simulink model "KUKA_Linear"  (R2020b)
settings: Solver=VariableStepAuto  StartTime=0.0  StopTime=200  RelTol=1e-3
(part 1 of 3)
settings Model: Creator=amin1  LastModifiedBy=amin1

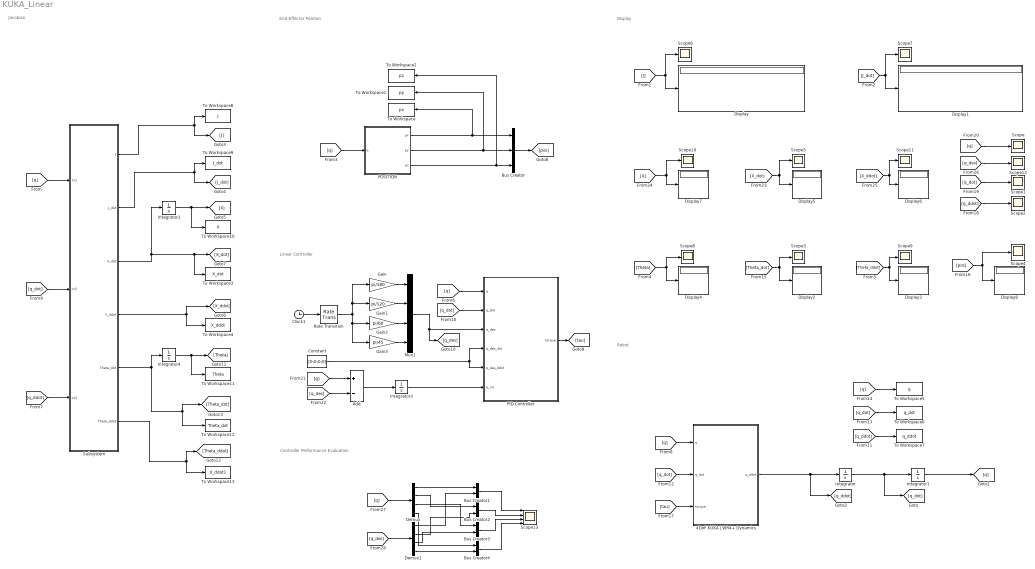
== system KUKA_Linear ==
  note: Controller Performance Evaluation
  note: Jacobian
  note: Display
  note: End-Effector Position
  note: Linear Controller
  note: Robot
  " 4DoF KUKA LWR4+ Dynamics" : MATLAB Function  TreatAsAtomicUnit=on
  Add : Sum  Inputs=+-
  Bus Creator : BusCreator  Inputs=3
  Bus Creator{1..4} (4 alike) : BusCreator  Inputs=2
  Clock1 : Clock
  Constant : Constant  Value=[0;0;0;0]
  Demux : Demux
  Demux1 : Demux
  Display{,1..8} (9 alike) : Display
  Gain : Gain  Gain=pi/180
  Gain1 : Gain  Gain=pi/120
  Gain2 : Gain  Gain=pi/60
  Gain3 : Gain  Gain=pi/45
  Integrator : Integrator  InitialCondition=[0;0;0;0]
  Integrator1 : Integrator  InitialCondition=[1;1;1;1]
  Integrator2 : Integrator  InitialCondition=[-0.458;-0.202;0.479]
  Integrator3 : Integrator  InitialCondition=[0;0;0;0]
  Integrator4 : Integrator  InitialCondition=[-0.455;-0.19;0.48]
  Mux1 : Mux
  PID Controller : MATLAB Function  TreatAsAtomicUnit=on
  POSITION : MATLAB Function  TreatAsAtomicUnit=on
  Rate Transition : RateTransition  OutPortSampleTime=10
  Scope{,1..12} (13 alike) : Scope
  Scope13 : Scope  NumInputPorts=4
  Subsystem : Subsystem
  To Workspace : ToWorkspace  VariableName=px  SampleTime=-1
  To Workspace1 : ToWorkspace  VariableName=py  SampleTime=-1
  To Workspace10 : ToWorkspace  VariableName=X  SampleTime=-1
  To Workspace11 : ToWorkspace  VariableName=Theta  SampleTime=-1
  To Workspace12 : ToWorkspace  VariableName=Theta_dot  SampleTime=-1
  To Workspace13 : ToWorkspace  VariableName=X_ddot1  SampleTime=-1
  To Workspace2 : ToWorkspace  VariableName=pz  SampleTime=-1
  To Workspace3 : ToWorkspace  VariableName=X_dot  SampleTime=-1
  To Workspace4 : ToWorkspace  VariableName=X_ddot  SampleTime=-1
  To Workspace5 : ToWorkspace  VariableName=q  SampleTime=-1
  To Workspace6 : ToWorkspace  VariableName=q_dot  SampleTime=-1
  To Workspace7 : ToWorkspace  VariableName=q_ddot  SampleTime=-1
  To Workspace8 : ToWorkspace  VariableName=J  SampleTime=-1
  To Workspace9 : ToWorkspace  VariableName=J_dot  SampleTime=-1
  wires:
  Gain/1 -> Mux1/1
  [q_dot] -> To Workspace6/1
  [q] -> To Workspace5/1
  POSITION/2(py) -> Bus Creator/2, To Workspace1/1
  Mux1/1 -> PID Controller/3(q_des), [q_des]
  Gain2/1 -> Mux1/3
  [q_dot] -> PID Controller/2(q_dot)
  [q_ddot] -> To Workspace7/1
  POSITION/3(pz) -> Bus Creator/3, To Workspace2/1
  Clock1/1 -> Rate Transition/1
  Constant/1 -> PID Controller/5(q_des_ddot), PID Controller/4(q_des_dot)
  [q] -> POSITION/1(q)
  [q] -> PID Controller/1(q)
  Rate Transition/1 -> Gain1/1, Gain/1, Gain2/1, Gain3/1
  " 4DoF KUKA LWR4+ Dynamics"/1(q_ddot) -> Integrator/1, [q_ddot]
  [q] -> " 4DoF KUKA LWR4+ Dynamics"/1(q)
  [q_dot] -> " 4DoF KUKA LWR4+ Dynamics"/2(q_dot)
  POSITION/1(px) -> Bus Creator/1, To Workspace/1
  Gain1/1 -> Mux1/2
  Integrator/1 -> Integrator1/1, [q_dot]
  Integrator1/1 -> [q]
  Gain3/1 -> Mux1/4
  Subsystem/2(J_dot) -> [J_dot], To Workspace9/1
  Subsystem/3(X_dot) -> Integrator2/1, To Workspace3/1, [X_dot]
  Subsystem/1(J) -> [J], To Workspace8/1
  [q] -> Subsystem/1(In1)
  [q_ddot] -> Subsystem/3(In3)
  [q_dot] -> Subsystem/2(In2)
  Subsystem/4(X_ddot) -> To Workspace4/1, [X_ddot]
  Integrator2/1 -> To Workspace10/1, [X]
  [J] -> Display/1, Scope6/1
  [J_dot] -> Display1/1, Scope7/1
  [Theta] -> Display4/1, Scope8/1
  [Theta_dot] -> Display2/1, Scope3/1
  [Theta_ddot] -> Display3/1, Scope9/1
  Bus Creator/1 -> [pos]
  [pos] -> Display8/1, Scope4/1
  PID Controller/1(torque) -> [tau]
  [tau] -> " 4DoF KUKA LWR4+ Dynamics"/3(torque)
  [q_ddot] -> Scope2/1
  [q_dot] -> Scope1/1
  [q] -> Scope/1
  [q] -> Add/1
  [q_des] -> Add/2
  Add/1 -> Integrator3/1
  Integrator3/1 -> PID Controller/6(e_int)
  Subsystem/5(Theta_dot) -> [Theta_dot], To Workspace12/1, Integrator4/1
  Integrator4/1 -> To Workspace11/1, [Theta]
  Subsystem/6(Theta_ddot) -> [Theta_ddot], To Workspace13/1
  [X_ddot] -> Display6/1, Scope11/1
  [X_dot] -> Display5/1, Scope5/1
  [X] -> Display7/1, Scope10/1
  [q_des] -> Scope12/1
  [q] -> Demux/1
  [q_des] -> Demux1/1
  Demux/1 -> Bus Creator1/1
  Demux1/1 -> Bus Creator1/2
  Demux/2 -> Bus Creator2/1
  Demux1/2 -> Bus Creator2/2
  Demux/3 -> Bus Creator3/1
  Demux1/3 -> Bus Creator3/2
  Demux/4 -> Bus Creator4/1
  Demux1/4 -> Bus Creator4/2
  Bus Creator1/1 -> Scope13/1
  Bus Creator2/1 -> Scope13/2
  Bus Creator3/1 -> Scope13/3
  Bus Creator4/1 -> Scope13/4

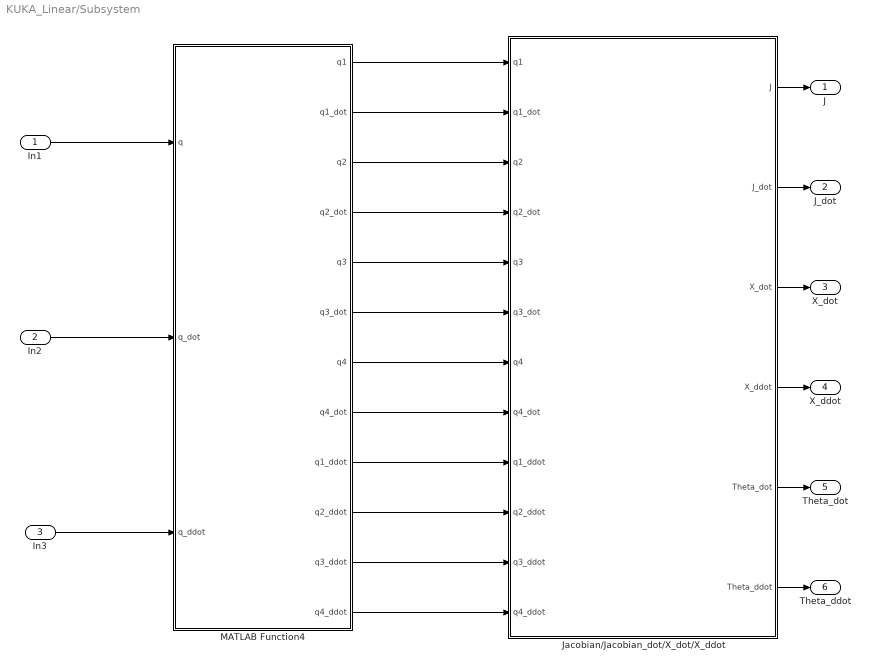
== system KUKA_Linear/Subsystem ==
  In1 : Inport
  In2 : Inport  Port=2
  In3 : Inport  Port=3
  Jacobian/Jacobian_dot/X_dot/X_ddot : MATLAB Function  TreatAsAtomicUnit=on
  MATLAB Function4 : MATLAB Function  TreatAsAtomicUnit=on
  J : Outport
  J_dot : Outport  Port=2
  X_dot : Outport  Port=3
  X_ddot : Outport  Port=4
  Theta_dot : Outport  Port=5
  Theta_ddot : Outport  Port=6
  wires:
  In2/1 -> MATLAB Function4/2(q_dot)
  In3/1 -> MATLAB Function4/3(q_ddot)
  In1/1 -> MATLAB Function4/1(q)
  MATLAB Function4/3(q2) -> Jacobian/Jacobian_dot/X_dot/X_ddot/3(q2)
  MATLAB Function4/10(q2_ddot) -> Jacobian/Jacobian_dot/X_dot/X_ddot/10(q2_ddot)
  MATLAB Function4/4(q2_dot) -> Jacobian/Jacobian_dot/X_dot/X_ddot/4(q2_dot)
  MATLAB Function4/11(q3_ddot) -> Jacobian/Jacobian_dot/X_dot/X_ddot/11(q3_ddot)
  MATLAB Function4/2(q1_dot) -> Jacobian/Jacobian_dot/X_dot/X_ddot/2(q1_dot)
  MATLAB Function4/1(q1) -> Jacobian/Jacobian_dot/X_dot/X_ddot/1(q1)
  MATLAB Function4/5(q3) -> Jacobian/Jacobian_dot/X_dot/X_ddot/5(q3)
  MATLAB Function4/6(q3_dot) -> Jacobian/Jacobian_dot/X_dot/X_ddot/6(q3_dot)
  MATLAB Function4/9(q1_ddot) -> Jacobian/Jacobian_dot/X_dot/X_ddot/9(q1_ddot)
  Jacobian/Jacobian_dot/X_dot/X_ddot/1(J) -> J/1
  Jacobian/Jacobian_dot/X_dot/X_ddot/2(J_dot) -> J_dot/1
  Jacobian/Jacobian_dot/X_dot/X_ddot/3(X_dot) -> X_dot/1
  Jacobian/Jacobian_dot/X_dot/X_ddot/4(X_ddot) -> X_ddot/1
  MATLAB Function4/7(q4) -> Jacobian/Jacobian_dot/X_dot/X_ddot/7(q4)
  MATLAB Function4/8(q4_dot) -> Jacobian/Jacobian_dot/X_dot/X_ddot/8(q4_dot)
  MATLAB Function4/12(q4_ddot) -> Jacobian/Jacobian_dot/X_dot/X_ddot/12(q4_ddot)
  Jacobian/Jacobian_dot/X_dot/X_ddot/6(Theta_ddot) -> Theta_ddot/1
  Jacobian/Jacobian_dot/X_dot/X_ddot/5(Theta_dot) -> Theta_dot/1

== matlab function KUKA_Linear/PID Controller ==
  data: q input; q_dot input; q_des input; torque output; q_des_dot input; q_des_ddot input; e_int input
function torque = fcn(q,q_dot,q_des,q_des_dot,q_des_ddot,e_int)
%#codegen

%% parameters
td1 = q_dot(1);
td2 = q_dot(2);
td3 = q_dot(3);
td4 = q_dot(4);

%% Constant
d3 = 0.4;

m1 = 2.7;
m2 = 2.7;
m3 = 2.7;
m4 = 2.7;

cx1 = 0.001340;
cx2 = 0.001340;
cx3 = -0.001340;
cx4 = -0.001340;

cy1 = -0.87777;
cy2 = -0.02622;
cy3 = 0.87777;
cy4 = 0.02622;

cz1 = -0.02622;
cz2 = 0.87777;
cz3 = -0.02622;
cz4 = 0.87777;

g = 9.8;

Ixx1 = 0.039; 
Ixy1 = 3.206e-4;
Ixz1 = 9.415e-5;
Iyy1 = 6.887e-3;
Iyz1 = -2.681e-3;
Izz1 = 0.03698;

Ixx2 = 0.039; 
Ixy2 = 9.415e-5;
Ixz2 = -3.145e-4;
Iyy2 = 0.03698;
Iyz2 = 9.747e-3;
Izz2 = 6.887e-3;

Ixx3 = 6.887e-3; 
Ixy3 = 3.145e-4;
Ixz3 = -9.5572e-5;
Iyy3 = 6.8872e-3;
Iyz3 = 2.681e-3;
Izz3 = 0.037;

Ixx4 = 0.037; 
Ixy4 = 9.415e-5;
Ixz4 = 3.1455e-4;
Iyy4 = 0.037;
Iyz4 = 9.747e-3;
Izz4 = 6.887e-3;

%% Triangle relative

c1 = cos(q(1));
c2 = cos(q(2));
c3 = cos(q(3));
c4 = cos(q(4)); 

s1 = sin(q(1));
s2 = sin(q(2));
s3 = sin(q(3));
s4 = sin(q(4));

%% matrix M

m11 = m1*cx1^2 + m1*cy1^2 + Izz1 - Iyz2*c2 - Ixz2*s2 - s2*(Ixz3*c2 + c3*(Ixx4*(c2*s4 - c3*c4*s2) - Ixy4*(c2*c4 + c3*s2*s4) + cy4*m4*(cy4*(c2*s4 - c3*c4*s2) - cx4*(c2*c4 + c3*s2*s4) + c3*d3*s2) + cz4*m4*(cz4*(c2*s4 - c3*c4*s2) - cx4*s2*s3 + d3*s2*s3*s4) - Ixz4*s2*s3) + s3*(Ixy4*(c2*s4 - c3*c4*s2) - Iyy4*(c2*c4 + c3*s2*s4) + cx4*m4*(cy4*(c2*s4 - c3*c4*s2) - cx4*(c2*c4 + c3*s2*s4) + c3*d3*s2) - cz4*m4*(cz4*(c2*c4 + c3*s2*s4) - cy4*s2*s3 + c4*d3*s2*s3) + Iyz4*s2*s3) - d3*m4*(cy4*(c2*s4 - c3*c4*s2) - cx4*(c2*c4 + c3*s2*s4) + c3*d3*s2) + cz3*m3*(c2*cx3 - c3*cz3*s2) - Ixx3*c3*s2 - Ixy3*s2*s3 - cy3*m3*(c3*cy3*s2 + cx3*s2*s3)) - c2*(Iyz3*c2 + d3*(c3*m4*(cz4*(c2*c4 + c3*s2*s4) - cy4*s2*s3 + c4*d3*s2*s3) + m4*s3*(cz4*(c2*s4 - c3*c4*s2) - cx4*s2*s3 + d3*s2*s3*s4)) - Ixz4*(c2*s4 - c3*c4*s2) - Iyz4*(c2*c4 + c3*s2*s4) - cy4*m4*(cz4*(c2*c4 + c3*s2*s4) - cy4*s2*s3 + c4*d3*s2*s3) - cx4*m4*(cz4*(c2*s4 - c3*c4*s2) - cx4*s2*s3 + d3*s2*s3*s4) + cz3*m3*(c2*cy3 + cz3*s2*s3) + Ixy3*c3*s2 + Iyy3*s2*s3 + Izz4*s2*s3 + cx3*m3*(c3*cy3*s2 + cx3*s2*s3)) - cx2*cz2*m2*s2 - c2*cy2*cz2*m2;
m12 = m2*cx2^2 + m2*cy2^2 + Izz2 - c2*(c3*m3*cz3^2 - d3*(c3*m4*(c3*cy4 - c3*c4*d3 + cz4*s3*s4) - m4*s3*(c4*cz4*s3 - c3*cx4 + c3*d3*s4)) + Iyy3*c3 + Izz4*c3 - Ixy3*s3 - Ixz4*c4*s3 + Iyz4*s3*s4 - cx4*m4*(c4*cz4*s3 - c3*cx4 + c3*d3*s4) + cy4*m4*(c3*cy4 - c3*c4*d3 + cz4*s3*s4) + cx3*m3*(c3*cx3 - cy3*s3)) - s2*(m3*s3*cz3^2 - Ixy3*c3 + Ixx3*s3 + c3*(cy4*m4*(c4*cy4*s3 - d3*s3 + cx4*s3*s4) - Ixz4*c3 + Ixx4*c4*s3 + Ixy4*s3*s4 + cz4*m4*(c4*cz4*s3 - c3*cx4 + c3*d3*s4)) + s3*(Iyz4*c3 + cx4*m4*(c4*cy4*s3 - d3*s3 + cx4*s3*s4) + Ixy4*c4*s3 + Iyy4*s3*s4 + cz4*m4*(c3*cy4 - c3*c4*d3 + cz4*s3*s4)) - d3*m4*(c4*cy4*s3 - d3*s3 + cx4*s3*s4) - cy3*m3*(c3*cx3 - cy3*s3));
m13 = c2*(Iyz4*c4 - Iyz3 + Ixz4*s4 - d3*(cz4*m4*s3*s4 + c3*c4*cz4*m4) - cy3*cz3*m3 + cx4*cz4*m4*s4 + c4*cy4*cz4*m4) - s2*(Ixz3 - c3*(- m4*s4*cz4^2 + Ixy4*c4 - Ixx4*s4 + cy4*m4*(c4*cx4 - cy4*s4)) - s3*(c4*m4*cz4^2 + Iyy4*c4 - Ixy4*s4 + cx4*m4*(c4*cx4 - cy4*s4)) + cx3*cz3*m3 + d3*m4*(c4*cx4 - cy4*s4));
m14 = s2*(s3*(Iyz4 + cy4*cz4*m4) - c3*(Ixz4 + cx4*cz4*m4)) + c2*(Izz4 - d3*(c3*cy4*m4 + cx4*m4*s3) + cx4^2*m4 + cy4^2*m4);

m21 = - Iyz2*c2 - Ixz2*s2 - s2*(Ixz3*c2 + c3*(Ixx4*(c2*s4 - c3*c4*s2) - Ixy4*(c2*c4 + c3*s2*s4) + cy4*m4*(cy4*(c2*s4 - c3*c4*s2) - cx4*(c2*c4 + c3*s2*s4) + c3*d3*s2) + cz4*m4*(cz4*(c2*s4 - c3*c4*s2) - cx4*s2*s3 + d3*s2*s3*s4) - Ixz4*s2*s3) + s3*(Ixy4*(c2*s4 - c3*c4*s2) - Iyy4*(c2*c4 + c3*s2*s4) + cx4*m4*(cy4*(c2*s4 - c3*c4*s2) - cx4*(c2*c4 + c3*s2*s4) + c3*d3*s2) - cz4*m4*(cz4*(c2*c4 + c3*s2*s4) - cy4*s2*s3 + c4*d3*s2*s3) + Iyz4*s2*s3) - d3*m4*(cy4*(c2*s4 - c3*c4*s2) - cx4*(c2*c4 + c3*s2*s4) + c3*d3*s2) + cz3*m3*(c2*cx3 - c3*cz3*s2) - Ixx3*c3*s2 - Ixy3*s2*s3 - cy3*m3*(c3*cy3*s2 + cx3*s2*s3)) - c2*(Iyz3*c2 + d3*(c3*m4*(cz4*(c2*c4 + c3*s2*s4) - cy4*s2*s3 + c4*d3*s2*s3) + m4*s3*(cz4*(c2*s4 - c3*c4*s2) - cx4*s2*s3 + d3*s2*s3*s4)) - Ixz4*(c2*s4 - c3*c4*s2) - Iyz4*(c2*c4 + c3*s2*s4) - cy4*m4*(cz4*(c2*c4 + c3*s2*s4) - cy4*s2*s3 + c4*d3*s2*s3) - cx4*m4*(cz4*(c2*s4 - c3*c4*s2) - cx4*s2*s3 + d3*s2*s3*s4) + cz3*m3*(c2*cy3 + cz3*s2*s3) + Ixy3*c3*s2 + Iyy3*s2*s3 + Izz4*s2*s3 + cx3*m3*(c3*cy3*s2 + cx3*s2*s3)) - cx2*cz2*m2*s2 - c2*cy2*cz2*m2;
m22 = m2*cx2^2 + m2*cy2^2 + Izz2 - c2*(c3*m3*cz3^2 - d3*(c3*m4*(c3*cy4 - c3*c4*d3 + cz4*s3*s4) - m4*s3*(c4*cz4*s3 - c3*cx4 + c3*d3*s4)) + Iyy3*c3 + Izz4*c3 - Ixy3*s3 - Ixz4*c4*s3 + Iyz4*s3*s4 - cx4*m4*(c4*cz4*s3 - c3*cx4 + c3*d3*s4) + cy4*m4*(c3*cy4 - c3*c4*d3 + cz4*s3*s4) + cx3*m3*(c3*cx3 - cy3*s3)) - s2*(m3*s3*cz3^2 - Ixy3*c3 + Ixx3*s3 + c3*(cy4*m4*(c4*cy4*s3 - d3*s3 + cx4*s3*s4) - Ixz4*c3 + Ixx4*c4*s3 + Ixy4*s3*s4 + cz4*m4*(c4*cz4*s3 - c3*cx4 + c3*d3*s4)) + s3*(Iyz4*c3 + cx4*m4*(c4*cy4*s3 - d3*s3 + cx4*s3*s4) + Ixy4*c4*s3 + Iyy4*s3*s4 + cz4*m4*(c3*cy4 - c3*c4*d3 + cz4*s3*s4)) - d3*m4*(c4*cy4*s3 - d3*s3 + cx4*s3*s4) - cy3*m3*(c3*cx3 - cy3*s3));
m23 = c2*(Iyz4*c4 - Iyz3 + Ixz4*s4 - d3*(cz4*m4*s3*s4 + c3*c4*cz4*m4) - cy3*cz3*m3 + cx4*cz4*m4*s4 + c4*cy4*cz4*m4) - s2*(Ixz3 - c3*(- m4*s4*cz4^2 + Ixy4*c4 - Ixx4*s4 + cy4*m4*(c4*cx4 - cy4*s4)) - s3*(c4*m4*cz4^2 + Iyy4*c4 - Ixy4*s4 + cx4*m4*(c4*cx4 - cy4*s4)) + cx3*cz3*m3 + d3*m4*(c4*cx4 - cy4*s4));
m24 = s2*(s3*(Iyz4 + cy4*cz4*m4) - c3*(Ixz4 + cx4*cz4*m4)) + c2*(Izz4 - d3*(c3*cy4*m4 + cx4*m4*s3) + cx4^2*m4 + cy4^2*m4);

m31 = Izz3*c2 - c3*(Ixy4*(c2*s4 - c3*c4*s2) - Iyy4*(c2*c4 + c3*s2*s4) + cx4*m4*(cy4*(c2*s4 - c3*c4*s2) - cx4*(c2*c4 + c3*s2*s4) + c3*d3*s2) - cz4*m4*(cz4*(c2*c4 + c3*s2*s4) - cy4*s2*s3 + c4*d3*s2*s3) + Iyz4*s2*s3) + s3*(Ixx4*(c2*s4 - c3*c4*s2) - Ixy4*(c2*c4 + c3*s2*s4) + cy4*m4*(cy4*(c2*s4 - c3*c4*s2) - cx4*(c2*c4 + c3*s2*s4) + c3*d3*s2) + cz4*m4*(cz4*(c2*s4 - c3*c4*s2) - cx4*s2*s3 + d3*s2*s3*s4) - Ixz4*s2*s3) + cx3*m3*(c2*cx3 - c3*cz3*s2) + cy3*m3*(c2*cy3 + cz3*s2*s3) - Ixz3*c3*s2 + Iyz3*s2*s3;
m32 = Iyz3*c3 + Ixz3*s3 - c3*(Iyz4*c3 + cx4*m4*(c4*cy4*s3 - d3*s3 + cx4*s3*s4) + Ixy4*c4*s3 + Iyy4*s3*s4 + cz4*m4*(c3*cy4 - c3*c4*d3 + cz4*s3*s4)) + s3*(cy4*m4*(c4*cy4*s3 - d3*s3 + cx4*s3*s4) - Ixz4*c3 + Ixx4*c4*s3 + Ixy4*s3*s4 + cz4*m4*(c4*cz4*s3 - c3*cx4 + c3*d3*s4)) + cx3*cz3*m3*s3 + c3*cy3*cz3*m3;
m33 = m3*cx3^2 + m3*cy3^2 + Izz3 + c3*(c4*m4*cz4^2 + Iyy4*c4 - Ixy4*s4 + cx4*m4*(c4*cx4 - cy4*s4)) - s3*(- m4*s4*cz4^2 + Ixy4*c4 - Ixx4*s4 + cy4*m4*(c4*cx4 - cy4*s4));
m34 = s3*(Ixz4 + cx4*cz4*m4) + c3*(Iyz4 + cy4*cz4*m4);

m41 = Ixz4*(c2*s4 - c3*c4*s2) + Iyz4*(c2*c4 + c3*s2*s4) + cy4*m4*(cz4*(c2*c4 + c3*s2*s4) - cy4*s2*s3 + c4*d3*s2*s3) + cx4*m4*(cz4*(c2*s4 - c3*c4*s2) - cx4*s2*s3 + d3*s2*s3*s4) - Izz4*s2*s3;
m42 = Ixz4*c4*s3 - Izz4*c3 - Iyz4*s3*s4 + cx4*m4*(c4*cz4*s3 - c3*cx4 + c3*d3*s4) - cy4*m4*(c3*cy4 - c3*c4*d3 + cz4*s3*s4);
m43 = Iyz4*c4 + Ixz4*s4 + cx4*cz4*m4*s4 + c4*cy4*cz4*m4;
m44 = m4*cx4^2 + m4*cy4^2 + Izz4;

M = [m11 m12 m13 m14;
     m21 m22 m23 m24;
     m31 m32 m33 m34;
     m41 m42 m43 m44];
 
%% matrix V

corio1 = (td2^2*(c2*(2*s3*(Iyz3*c3 + Ixz3*s3) - d3*(c3*m4*(2*c3*(c3*cx4 - c4*cz4*s3) - s4*(2*d3*c3^2 + 2*d3*s3^2) + 2*s3*s4*(c4*cy4*s3 + cx4*s3*s4)) - m4*s3*(2*c3*(c3*cy4 + cz4*s3*s4) - c4*(2*d3*c3^2 + 2*d3*s3^2) + 2*c4*s3*(c4*cy4*s3 + cx4*s3*s4))) - cx4*m4*(2*c3*(c3*cy4 + cz4*s3*s4) - c4*(2*d3*c3^2 + 2*d3*s3^2) + 2*c4*s3*(c4*cy4*s3 + cx4*s3*s4)) + cy4*m4*(2*c3*(c3*cx4 - c4*cz4*s3) - s4*(2*d3*c3^2 + 2*d3*s3^2) + 2*s3*s4*(c4*cy4*s3 + cx4*s3*s4)) + cx3*m3*(2*cz3*c3^2 + 2*cz3*s3^2) - 2*c4*s3*(Iyz4*c3 + Ixy4*c4*s3 + Iyy4*s3*s4) + 2*s3*s4*(Ixx4*c4*s3 - Ixz4*c3 + Ixy4*s3*s4) - 2*c3*cz3*m3*(c3*cx3 - cy3*s3)) - s2*(2*c3*(Iyz3*c3 + Ixz3*s3) - s3*(cx4*m4*(2*c4*s3*(c3*cx4 - c4*cz4*s3) - 2*s3*s4*(c3*cy4 + cz4*s3*s4)) - 2*c3*(Ixx4*c4*s3 - Ixz4*c3 + Ixy4*s3*s4) + cz4*m4*(2*c3*(c3*cx4 - c4*cz4*s3) - s4*(2*d3*c3^2 + 2*d3*s3^2) + 2*s3*s4*(c4*cy4*s3 + cx4*s3*s4)) + 2*c4*s3*(Izz4*c3 - Ixz4*c4*s3 + Iyz4*s3*s4)) - c3*(2*c3*(Iyz4*c3 + Ixy4*c4*s3 + Iyy4*s3*s4) + cy4*m4*(2*c4*s3*(c3*cx4 - c4*cz4*s3) - 2*s3*s4*(c3*cy4 + cz4*s3*s4)) + cz4*m4*(2*c3*(c3*cy4 + cz4*s3*s4) - c4*(2*d3*c3^2 + 2*d3*s3^2) + 2*c4*s3*(c4*cy4*s3 + cx4*s3*s4)) - 2*s3*s4*(Izz4*c3 - Ixz4*c4*s3 + Iyz4*s3*s4)) + d3*m4*(2*c4*s3*(c3*cx4 - c4*cz4*s3) - 2*s3*s4*(c3*cy4 + cz4*s3*s4)) + cy3*m3*(2*cz3*c3^2 + 2*cz3*s3^2) + 2*cz3*m3*s3*(c3*cx3 - cy3*s3))))/2 + (td3^2*(s2*(2*Iyz3 - c3*(2*c4*(Iyz4*c4 + Ixz4*s4) + cy4*m4*(2*cz4*c4^2 + 2*cz4*s4^2) + 2*cz4*m4*s4*(c4*cx4 - cy4*s4)) - s3*(2*s4*(Iyz4*c4 + Ixz4*s4) + cx4*m4*(2*cz4*c4^2 + 2*cz4*s4^2) - 2*c4*cz4*m4*(c4*cx4 - cy4*s4)) + 2*cy3*cz3*m3 + d3*m4*(2*cz4*c4^2 + 2*cz4*s4^2)) + c2*(2*c4*(Ixy4*c4 - Ixx4*s4) - 2*Ixz3 + 2*s4*(Iyy4*c4 - Ixy4*s4) - d3*(2*c3*c4*m4*(c4*cx4 - cy4*s4) + 2*m4*s3*s4*(c4*cx4 - cy4*s4)) - 2*cx3*cz3*m3 + 2*c4*cy4*m4*(c4*cx4 - cy4*s4) + 2*cx4*m4*s4*(c4*cx4 - cy4*s4))))/2 + (td4^2*(s2*(c3*(2*Iyz4 + 2*cy4*cz4*m4) + s3*(2*Ixz4 + 2*cx4*cz4*m4)) - c2*d3*(2*c3*cx4*m4 - 2*cy4*m4*s3)))/2 + (td1^2*(s2*(2*c2*(Iyz3*c2 + Ixy3*c3*s2 + Iyy3*s2*s3) - c3*(2*(c2*c4 + c3*s2*s4)*(Ixz4*(c2*s4 - c3*c4*s2) + Iyz4*(c2*c4 + c3*s2*s4) - Izz4*s2*s3) + cy4*m4*(2*(c2*s4 - c3*c4*s2)*(cz4*(c2*s4 - c3*c4*s2) - cx4*s2*s3) + 2*(c2*c4 + c3*s2*s4)*(cz4*(c2*c4 + c3*s2*s4) - cy4*s2*s3) + 2*c2*d3*s2*s3) - 2*s2*s3*(Ixy4*(c2*s4 - c3*c4*s2) - Iyy4*(c2*c4 + c3*s2*s4) + Iyz4*s2*s3) + cz4*m4*(2*(c2*s4 - c3*c4*s2)*(cx4*(c2*c4 + c3*s2*s4) - cy4*(c2*s4 - c3*c4*s2)) + c4*(2*d3*c3^2*s2^2 + 2*d3*s2^2*s3^2) + 2*s2*s3*(cz4*(c2*c4 + c3*s2*s4) - cy4*s2*s3) - 2*c2*c3*d3*s2*s4)) - s3*(2*(c2*s4 - c3*c4*s2)*(Ixz4*(c2*s4 - c3*c4*s2) + Iyz4*(c2*c4 + c3*s2*s4) - Izz4*s2*s3) + cx4*m4*(2*(c2*s4 - c3*c4*s2)*(cz4*(c2*s4 - c3*c4*s2) - cx4*s2*s3) + 2*(c2*c4 + c3*s2*s4)*(cz4*(c2*c4 + c3*s2*s4) - cy4*s2*s3) + 2*c2*d3*s2*s3) - 2*s2*s3*(Ixy4*(c2*c4 + c3*s2*s4) - Ixx4*(c2*s4 - c3*c4*s2) + Ixz4*s2*s3) + cz4*m4*(s4*(2*d3*c3^2*s2^2 + 2*d3*s2^2*s3^2) - 2*(c2*c4 + c3*s2*s4)*(cx4*(c2*c4 + c3*s2*s4) - cy4*(c2*s4 - c3*c4*s2)) + 2*s2*s3*(cz4*(c2*s4 - c3*c4*s2) - cx4*s2*s3) + 2*c2*c3*c4*d3*s2)) + cz3*m3*(2*c2*(c2*cy3 + cz3*s2*s3) + 2*c3*s2*(c3*cy3*s2 + cx3*s2*s3)) + cy3*m3*(2*c3*s2*(c2*cx3 - c3*cz3*s2) - 2*s2*s3*(c2*cy3 + cz3*s2*s3)) + d3*m4*(2*(c2*s4 - c3*c4*s2)*(cz4*(c2*s4 - c3*c4*s2) - cx4*s2*s3) + 2*(c2*c4 + c3*s2*s4)*(cz4*(c2*c4 + c3*s2*s4) - cy4*s2*s3) + 2*c2*d3*s2*s3) - 2*s2*s3*(Izz3*c2 - Ixz3*c3*s2 + Iyz3*s2*s3)) + 2*c2*(Ixy2*c2 - Ixx2*s2) + 2*s2*(Iyy2*c2 - Ixy2*s2) - c2*(2*(c2*s4 - c3*c4*s2)*(Ixy4*(c2*s4 - c3*c4*s2) - Iyy4*(c2*c4 + c3*s2*s4) + Iyz4*s2*s3) - 2*(c2*c4 + c3*s2*s4)*(Ixy4*(c2*c4 + c3*s2*s4) - Ixx4*(c2*s4 - c3*c4*s2) + Ixz4*s2*s3) - d3*(c3*m4*(s4*(2*d3*c3^2*s2^2 + 2*d3*s2^2*s3^2) - 2*(c2*c4 + c3*s2*s4)*(cx4*(c2*c4 + c3*s2*s4) - cy4*(c2*s4 - c3*c4*s2)) + 2*s2*s3*(cz4*(c2*s4 - c3*c4*s2) - cx4*s2*s3) + 2*c2*c3*c4*d3*s2) - m4*s3*(2*(c2*s4 - c3*c4*s2)*(cx4*(c2*c4 + c3*s2*s4) - cy4*(c2*s4 - c3*c4*s2)) + c4*(2*d3*c3^2*s2^2 + 2*d3*s2^2*s3^2) + 2*s2*s3*(cz4*(c2*c4 + c3*s2*s4) - cy4*s2*s3) - 2*c2*c3*d3*s2*s4)) - 2*c2*(Ixx3*c3*s2 - Ixz3*c2 + Ixy3*s2*s3) + cx3*m3*(2*c3*s2*(c2*cx3 - c3*cz3*s2) - 2*s2*s3*(c2*cy3 + cz3*s2*s3)) + cz3*m3*(2*c2*(c2*cx3 - c3*cz3*s2) + 2*s2*s3*(c3*cy3*s2 + cx3*s2*s3)) + 2*c3*s2*(Izz3*c2 - Ixz3*c3*s2 + Iyz3*s2*s3) - cx4*m4*(2*(c2*s4 - c3*c4*s2)*(cx4*(c2*c4 + c3*s2*s4) - cy4*(c2*s4 - c3*c4*s2)) + c4*(2*d3*c3^2*s2^2 + 2*d3*s2^2*s3^2) + 2*s2*s3*(cz4*(c2*c4 + c3*s2*s4) - cy4*s2*s3) - 2*c2*c3*d3*s2*s4) + cy4*m4*(s4*(2*d3*c3^2*s2^2 + 2*d3*s2^2*s3^2) - 2*(c2*c4 + c3*s2*s4)*(cx4*(c2*c4 + c3*s2*s4) - cy4*(c2*s4 - c3*c4*s2)) + 2*s2*s3*(cz4*(c2*s4 - c3*c4*s2) - cx4*s2*s3) + 2*c2*c3*c4*d3*s2)) + 2*c2*cy2*m2*(c2*cx2 - cy2*s2) + 2*cx2*m2*s2*(c2*cx2 - cy2*s2)))/2 - td2*td4*(s2*(s3*(2*Ixz4*c3 - Ixx4*c4*s3 + Iyy4*c4*s3 + Izz4*c4*s3 - 2*Ixy4*s3*s4 + cx4*m4*(2*c4*cx4*s3 - 2*cy4*s3*s4) + 2*c3*cx4*cz4*m4) + c3*(2*Iyz4*c3 + 2*Ixy4*c4*s3 - Ixx4*s3*s4 + Iyy4*s3*s4 - Izz4*s3*s4 + cy4*m4*(2*c4*cx4*s3 - 2*cy4*s3*s4) + 2*c3*cy4*cz4*m4) - d3*m4*(2*c4*cx4*s3 - 2*cy4*s3*s4)) - c2*d3*(2*c3^2*cx4*m4 - 2*c3*cy4*m4*s3)) - td1*td3*(c2*(2*Ixz3*c2 - (c2*c4 + c3*s2*s4)*(Ixy4*c4 - Ixx4*s4) - (c2*s4 - c3*c4*s2)*(Iyy4*c4 - Ixy4*s4) + d3*(c3*m4*(c4*(cx4*(c2*c4 + c3*s2*s4) - cy4*(c2*s4 - c3*c4*s2)) + (c2*c4 + c3*s2*s4)*(c4*cx4 - cy4*s4) - c3*cy4*s2 - 2*cz4*s2*s3*s4) + m4*s3*(s4*(cx4*(c2*c4 + c3*s2*s4) - cy4*(c2*s4 - c3*c4*s2)) + (c2*s4 - c3*c4*s2)*(c4*cx4 - cy4*s4) - c3*cx4*s2 + 2*c4*cz4*s2*s3)) - c4*(Ixy4*(c2*c4 + c3*s2*s4) - Ixx4*(c2*s4 - c3*c4*s2) + Ixz4*s2*s3) + s4*(Ixy4*(c2*s4 - c3*c4*s2) - Iyy4*(c2*c4 + c3*s2*s4) + Iyz4*s2*s3) - Ixx3*c3*s2 + Iyy3*c3*s2 + Izz3*c3*s2 + Izz4*c3*s2 - cx4*m4*(s4*(cx4*(c2*c4 + c3*s2*s4) - cy4*(c2*s4 - c3*c4*s2)) + (c2*s4 - c3*c4*s2)*(c4*cx4 - cy4*s4) - c3*cx4*s2 + 2*c4*cz4*s2*s3) - cy4*m4*(c4*(cx4*(c2*c4 + c3*s2*s4) - cy4*(c2*s4 - c3*c4*s2)) + (c2*c4 + c3*s2*s4)*(c4*cx4 - cy4*s4) - c3*cy4*s2 - 2*cz4*s2*s3*s4) - 2*Ixy3*s2*s3 + cx3*m3*(2*c3*cx3*s2 - 2*cy3*s2*s3) + Iyz4*s2*s3*s4 - Ixz4*c4*s2*s3 + 2*c2*cx3*cz3*m3) - s2*(2*Iyz3*c2 - c3*((c2*c4 + c3*s2*s4)*(Iyz4*c4 + Ixz4*s4) + c4*(Ixz4*(c2*s4 - c3*c4*s2) + Iyz4*(c2*c4 + c3*s2*s4) - Izz4*s2*s3) - Ixz4*c3*s2 + cz4*m4*(s4*(cx4*(c2*c4 + c3*s2*s4) - cy4*(c2*s4 - c3*c4*s2)) + (c2*s4 - c3*c4*s2)*(c4*cx4 - cy4*s4) - c3*cx4*s2 + 2*c4*cz4*s2*s3) + s2*s3*(Iyy4*c4 - Ixy4*s4) + cy4*m4*(c4*(cz4*(c2*c4 + c3*s2*s4) - cy4*s2*s3) + s4*(cz4*(c2*s4 - c3*c4*s2) - cx4*s2*s3) + c4*cz4*(c2*c4 + c3*s2*s4) + cz4*s4*(c2*s4 - c3*c4*s2) + c4*cy4*s2*s3 + cx4*s2*s3*s4) + Ixy4*s2*s3*s4 + Ixx4*c4*s2*s3) - s3*((c2*s4 - c3*c4*s2)*(Iyz4*c4 + Ixz4*s4) + s4*(Ixz4*(c2*s4 - c3*c4*s2) + Iyz4*(c2*c4 + c3*s2*s4) - Izz4*s2*s3) + Iyz4*c3*s2 - cz4*m4*(c4*(cx4*(c2*c4 + c3*s2*s4) - cy4*(c2*s4 - c3*c4*s2)) + (c2*c4 + c3*s2*s4)*(c4*cx4 - cy4*s4) - c3*cy4*s2 - 2*cz4*s2*s3*s4) - s2*s3*(Ixy4*c4 - Ixx4*s4) + cx4*m4*(c4*(cz4*(c2*c4 + c3*s2*s4) - cy4*s2*s3) + s4*(cz4*(c2*s4 - c3*c4*s2) - cx4*s2*s3) + c4*cz4*(c2*c4 + c3*s2*s4) + cz4*s4*(c2*s4 - c3*c4*s2) + c4*cy4*s2*s3 + cx4*s2*s3*s4) + Iyy4*s2*s3*s4 + Ixy4*c4*s2*s3) + 2*Ixy3*c3*s2 - Ixx3*s2*s3 + Iyy3*s2*s3 - Izz3*s2*s3 + cy3*m3*(2*c3*cx3*s2 - 2*cy3*s2*s3) + d3*m4*(c4*(cz4*(c2*c4 + c3*s2*s4) - cy4*s2*s3) + s4*(cz4*(c2*s4 - c3*c4*s2) - cx4*s2*s3) + c4*cz4*(c2*c4 + c3*s2*s4) + cz4*s4*(c2*s4 - c3*c4*s2) + c4*cy4*s2*s3 + cx4*s2*s3*s4) + 2*c2*cy3*cz3*m3)) - td1*td4*(s2*(s3*(2*Ixy4*(c2*c4 + c3*s2*s4) - Ixx4*(c2*s4 - c3*c4*s2) + Iyy4*(c2*s4 - c3*c4*s2) + Izz4*(c2*s4 - c3*c4*s2) + cx4*m4*(2*cx4*(c2*s4 - c3*c4*s2) + 2*cy4*(c2*c4 + c3*s2*s4)) + 2*Ixz4*s2*s3 + 2*cx4*cz4*m4*s2*s3) + c3*(Ixx4*(c2*c4 + c3*s2*s4) + 2*Ixy4*(c2*s4 - c3*c4*s2) - Iyy4*(c2*c4 + c3*s2*s4) + Izz4*(c2*c4 + c3*s2*s4) + cy4*m4*(2*cx4*(c2*s4 - c3*c4*s2) + 2*cy4*(c2*c4 + c3*s2*s4)) + 2*Iyz4*s2*s3 + 2*cy4*cz4*m4*s2*s3) - d3*m4*(2*cx4*(c2*s4 - c3*c4*s2) + 2*cy4*(c2*c4 + c3*s2*s4))) + c2*d3*(2*cy4*m4*s2*s3^2 - 2*c3*cx4*m4*s2*s3)) - td2*td3*(s2*(Ixx3*c3 - Iyy3*c3 + Izz3*c3 + 2*Ixy3*s3 + c3*(Ixz4*s3 - c4*(Izz4*c3 - Ixz4*c4*s3 + Iyz4*s3*s4) + c3*(Iyy4*c4 - Ixy4*s4) + Ixx4*c3*c4 + Ixy4*c3*s4 - cy4*m4*(s4*(c3*cx4 - c4*cz4*s3) + c4*(c3*cy4 + cz4*s3*s4) - c3*c4*cy4 - c3*cx4*s4) + cz4*m4*(cx4*s3 - s4*(c4*cy4*s3 + cx4*s3*s4) + 2*c3*c4*cz4 + c4*s3*(c4*cx4 - cy4*s4)) - s3*s4*(Iyz4*c4 + Ixz4*s4)) - s3*(Iyz4*s3 + c3*(Ixy4*c4 - Ixx4*s4) + s4*(Izz4*c3 - Ixz4*c4*s3 + Iyz4*s3*s4) - Ixy4*c3*c4 - Iyy4*c3*s4 + cx4*m4*(s4*(c3*cx4 - c4*cz4*s3) + c4*(c3*cy4 + cz4*s3*s4) - c3*c4*cy4 - c3*cx4*s4) - c4*s3*(Iyz4*c4 + Ixz4*s4) - cz4*m4*(c4*(c4*cy4*s3 + cx4*s3*s4) - cy4*s3 + s3*s4*(c4*cx4 - cy4*s4) + 2*c3*cz4*s4)) + d3*m4*(s4*(c3*cx4 - c4*cz4*s3) + c4*(c3*cy4 + cz4*s3*s4) - c3*c4*cy4 - c3*cx4*s4) + cy3*m3*(2*c3*cy3 + 2*cx3*s3)) - c2*(2*Ixy3*c3 - Ixx3*s3 + Iyy3*s3 + Izz3*s3 + Izz4*s3 - c4*(Ixx4*c4*s3 - Ixz4*c3 + Ixy4*s3*s4) - s4*(Iyz4*c3 + Ixy4*c4*s3 + Iyy4*s3*s4) - d3*(m4*s3*(cx4*s3 - s4*(c4*cy4*s3 + cx4*s3*s4) + 2*c3*c4*cz4 + c4*s3*(c4*cx4 - cy4*s4)) - c3*m4*(c4*(c4*cy4*s3 + cx4*s3*s4) - cy4*s3 + s3*s4*(c4*cx4 - cy4*s4) + 2*c3*cz4*s4)) + Ixz4*c3*c4 - Iyz4*c3*s4 + cx4*m4*(cx4*s3 - s4*(c4*cy4*s3 + cx4*s3*s4) + 2*c3*c4*cz4 + c4*s3*(c4*cx4 - cy4*s4)) + c4*s3*(Iyy4*c4 - Ixy4*s4) - cy4*m4*(c4*(c4*cy4*s3 + cx4*s3*s4) - cy4*s3 + s3*s4*(c4*cx4 - cy4*s4) + 2*c3*cz4*s4) - s3*s4*(Ixy4*c4 - Ixx4*s4) + cx3*m3*(2*c3*cy3 + 2*cx3*s3))) - td1*td2*(c2*((c2*c4 + c3*s2*s4)*(Ixx4*c4*s3 - Ixz4*c3 + Ixy4*s3*s4) + (c2*s4 - c3*c4*s2)*(Iyz4*c3 + Ixy4*c4*s3 + Iyy4*s3*s4) - d3*(m4*s3*((c2*s4 - c3*c4*s2)*(c4*cy4*s3 + cx4*s3*s4) - c3*(cz4*(c2*c4 + c3*s2*s4) - cy4*s2*s3) + cz4*(s2*s4 + c2*c3*c4) + s2*s3*(c3*cy4 + cz4*s3*s4) - c4*s3*(cx4*(c2*c4 + c3*s2*s4) - cy4*(c2*s4 - c3*c4*s2)) + c2*cx4*s3 - 2*c2*d3*s3*s4) + c3*m4*((c2*c4 + c3*s2*s4)*(c4*cy4*s3 + cx4*s3*s4) + c3*(cz4*(c2*s4 - c3*c4*s2) - cx4*s2*s3) + cz4*(c4*s2 - c2*c3*s4) - s2*s3*(c3*cx4 - c4*cz4*s3) + s3*s4*(cx4*(c2*c4 + c3*s2*s4) - cy4*(c2*s4 - c3*c4*s2)) + c2*cy4*s3 - 2*c2*c4*d3*s3)) - Iyz3*s2 - c2*(Ixy3*c3 - Ixx3*s3) - s3*(Izz3*c2 - Ixz3*c3*s2 + Iyz3*s2*s3) + Ixz4*(s2*s4 + c2*c3*c4) + Iyz4*(c4*s2 - c2*c3*s4) + Ixy3*c2*c3 + Iyy3*c2*s3 + Izz4*c2*s3 - cx3*m3*(s3*(c2*cx3 - c3*cz3*s2) + c3*(c2*cy3 + cz3*s2*s3) - c2*c3*cy3 - c2*cx3*s3) + c3*s2*(Iyz3*c3 + Ixz3*s3) + cz3*m3*(c3*(c3*cy3*s2 + cx3*s2*s3) - cy3*s2 + s2*s3*(c3*cx3 - cy3*s3) + 2*c2*cz3*s3) + c4*s3*(Ixy4*(c2*s4 - c3*c4*s2) - Iyy4*(c2*c4 + c3*s2*s4) + Iyz4*s2*s3) + s3*s4*(Ixy4*(c2*c4 + c3*s2*s4) - Ixx4*(c2*s4 - c3*c4*s2) + Ixz4*s2*s3) + cy4*m4*((c2*c4 + c3*s2*s4)*(c4*cy4*s3 + cx4*s3*s4) + c3*(cz4*(c2*s4 - c3*c4*s2) - cx4*s2*s3) + cz4*(c4*s2 - c2*c3*s4) - s2*s3*(c3*cx4 - c4*cz4*s3) + s3*s4*(cx4*(c2*c4 + c3*s2*s4) - cy4*(c2*s4 - c3*c4*s2)) + c2*cy4*s3 - 2*c2*c4*d3*s3) + cx4*m4*((c2*s4 - c3*c4*s2)*(c4*cy4*s3 + cx4*s3*s4) - c3*(cz4*(c2*c4 + c3*s2*s4) - cy4*s2*s3) + cz4*(s2*s4 + c2*c3*c4) + s2*s3*(c3*cy4 + cz4*s3*s4) - c4*s3*(cx4*(c2*c4 + c3*s2*s4) - cy4*(c2*s4 - c3*c4*s2)) + c2*cx4*s3 - 2*c2*d3*s3*s4)) - s2*(c3*((c2*c4 + c3*s2*s4)*(Izz4*c3 - Ixz4*c4*s3 + Iyz4*s3*s4) + c3*(Ixy4*(c2*s4 - c3*c4*s2) - Iyy4*(c2*c4 + c3*s2*s4) + Iyz4*s2*s3) + Ixx4*(s2*s4 + c2*c3*c4) - Ixy4*(c4*s2 - c2*c3*s4) + Ixz4*c2*s3 + s2*s3*(Iyz4*c3 + Ixy4*c4*s3 + Iyy4*s3*s4) + cy4*m4*((c3*cx4 - c4*cz4*s3)*(c2*s4 - c3*c4*s2) + (c2*c4 + c3*s2*s4)*(c3*cy4 + cz4*s3*s4) - cx4*(c4*s2 - c2*c3*s4) + cy4*(s2*s4 + c2*c3*c4) - c4*s3*(cz4*(c2*s4 - c3*c4*s2) - cx4*s2*s3) + s3*s4*(cz4*(c2*c4 + c3*s2*s4) - cy4*s2*s3) - 2*c2*c3*d3) + s3*s4*(Ixz4*(c2*s4 - c3*c4*s2) + Iyz4*(c2*c4 + c3*s2*s4) - Izz4*s2*s3) + cz4*m4*((c2*s4 - c3*c4*s2)*(c4*cy4*s3 + cx4*s3*s4) - c3*(cz4*(c2*c4 + c3*s2*s4) - cy4*s2*s3) + cz4*(s2*s4 + c2*c3*c4) + s2*s3*(c3*cy4 + cz4*s3*s4) - c4*s3*(cx4*(c2*c4 + c3*s2*s4) - cy4*(c2*s4 - c3*c4*s2)) + c2*cx4*s3 - 2*c2*d3*s3*s4)) - s3*(Iyy4*(c4*s2 - c2*c3*s4) - c3*(Ixy4*(c2*c4 + c3*s2*s4) - Ixx4*(c2*s4 - c3*c4*s2) + Ixz4*s2*s3) - Ixy4*(s2*s4 + c2*c3*c4) - (c2*s4 - c3*c4*s2)*(Izz4*c3 - Ixz4*c4*s3 + Iyz4*s3*s4) + Iyz4*c2*s3 + s2*s3*(Ixx4*c4*s3 - Ixz4*c3 + Ixy4*s3*s4) - cx4*m4*((c3*cx4 - c4*cz4*s3)*(c2*s4 - c3*c4*s2) + (c2*c4 + c3*s2*s4)*(c3*cy4 + cz4*s3*s4) - cx4*(c4*s2 - c2*c3*s4) + cy4*(s2*s4 + c2*c3*c4) - c4*s3*(cz4*(c2*s4 - c3*c4*s2) - cx4*s2*s3) + s3*s4*(cz4*(c2*c4 + c3*s2*s4) - cy4*s2*s3) - 2*c2*c3*d3) + c4*s3*(Ixz4*(c2*s4 - c3*c4*s2) + Iyz4*(c2*c4 + c3*s2*s4) - Izz4*s2*s3) + cz4*m4*((c2*c4 + c3*s2*s4)*(c4*cy4*s3 + cx4*s3*s4) + c3*(cz4*(c2*s4 - c3*c4*s2) - cx4*s2*s3) + cz4*(c4*s2 - c2*c3*s4) - s2*s3*(c3*cx4 - c4*cz4*s3) + s3*s4*(cx4*(c2*c4 + c3*s2*s4) - cy4*(c2*s4 - c3*c4*s2)) + c2*cy4*s3 - 2*c2*c4*d3*s3)) + Ixz3*s2 - c3*(Izz3*c2 - Ixz3*c3*s2 + Iyz3*s2*s3) + c2*(Iyy3*c3 - Ixy3*s3) + Ixx3*c2*c3 + Ixy3*c2*s3 - cy3*m3*(s3*(c2*cx3 - c3*cz3*s2) + c3*(c2*cy3 + cz3*s2*s3) - c2*c3*cy3 - c2*cx3*s3) + cz3*m3*(cx3*s2 - s3*(c3*cy3*s2 + cx3*s2*s3) + 2*c2*c3*cz3 + c3*s2*(c3*cx3 - cy3*s3)) - d3*m4*((c3*cx4 - c4*cz4*s3)*(c2*s4 - c3*c4*s2) + (c2*c4 + c3*s2*s4)*(c3*cy4 + cz4*s3*s4) - cx4*(c4*s2 - c2*c3*s4) + cy4*(s2*s4 + c2*c3*c4) - c4*s3*(cz4*(c2*s4 - c3*c4*s2) - cx4*s2*s3) + s3*s4*(cz4*(c2*c4 + c3*s2*s4) - cy4*s2*s3) - 2*c2*c3*d3) - s2*s3*(Iyz3*c3 + Ixz3*s3))) - s2*td3*td4*(c3*(Ixx4*c4 - Iyy4*c4 + Izz4*c4 + 2*Ixy4*s4 + cy4*m4*(2*c4*cy4 + 2*cx4*s4)) + s3*(2*Ixy4*c4 - Ixx4*s4 + Iyy4*s4 + Izz4*s4 + cx4*m4*(2*c4*cy4 + 2*cx4*s4)) - d3*m4*(2*c4*cy4 + 2*cx4*s4));
corio2 = (td2^2*(c2*(2*s3*(Iyz3*c3 + Ixz3*s3) - d3*(c3*m4*(2*c3*(c3*cx4 - c4*cz4*s3) - s4*(2*d3*c3^2 + 2*d3*s3^2) + 2*s3*s4*(c4*cy4*s3 + cx4*s3*s4)) - m4*s3*(2*c3*(c3*cy4 + cz4*s3*s4) - c4*(2*d3*c3^2 + 2*d3*s3^2) + 2*c4*s3*(c4*cy4*s3 + cx4*s3*s4))) - cx4*m4*(2*c3*(c3*cy4 + cz4*s3*s4) - c4*(2*d3*c3^2 + 2*d3*s3^2) + 2*c4*s3*(c4*cy4*s3 + cx4*s3*s4)) + cy4*m4*(2*c3*(c3*cx4 - c4*cz4*s3) - s4*(2*d3*c3^2 + 2*d3*s3^2) + 2*s3*s4*(c4*cy4*s3 + cx4*s3*s4)) + cx3*m3*(2*cz3*c3^2 + 2*cz3*s3^2) - 2*c4*s3*(Iyz4*c3 + Ixy4*c4*s3 + Iyy4*s3*s4) + 2*s3*s4*(Ixx4*c4*s3 - Ixz4*c3 + Ixy4*s3*s4) - 2*c3*cz3*m3*(c3*cx3 - cy3*s3)) - s2*(2*c3*(Iyz3*c3 + Ixz3*s3) - s3*(cx4*m4*(2*c4*s3*(c3*cx4 - c4*cz4*s3) - 2*s3*s4*(c3*cy4 + cz4*s3*s4)) - 2*c3*(Ixx4*c4*s3 - Ixz4*c3 + Ixy4*s3*s4) + cz4*m4*(2*c3*(c3*cx4 - c4*cz4*s3) - s4*(2*d3*c3^2 + 2*d3*s3^2) + 2*s3*s4*(c4*cy4*s3 + cx4*s3*s4)) + 2*c4*s3*(Izz4*c3 - Ixz4*c4*s3 + Iyz4*s3*s4)) - c3*(2*c3*(Iyz4*c3 + Ixy4*c4*s3 + Iyy4*s3*s4) + cy4*m4*(2*c4*s3*(c3*cx4 - c4*cz4*s3) - 2*s3*s4*(c3*cy4 + cz4*s3*s4)) + cz4*m4*(2*c3*(c3*cy4 + cz4*s3*s4) - c4*(2*d3*c3^2 + 2*d3*s3^2) + 2*c4*s3*(c4*cy4*s3 + cx4*s3*s4)) - 2*s3*s4*(Izz4*c3 - Ixz4*c4*s3 + Iyz4*s3*s4)) + d3*m4*(2*c4*s3*(c3*cx4 - c4*cz4*s3) - 2*s3*s4*(c3*cy4 + cz4*s3*s4)) + cy3*m3*(2*cz3*c3^2 + 2*cz3*s3^2) + 2*cz3*m3*s3*(c3*cx3 - cy3*s3))))/2 + (td3^2*(s2*(2*Iyz3 - c3*(2*c4*(Iyz4*c4 + Ixz4*s4) + cy4*m4*(2*cz4*c4^2 + 2*cz4*s4^2) + 2*cz4*m4*s4*(c4*cx4 - cy4*s4)) - s3*(2*s4*(Iyz4*c4 + Ixz4*s4) + cx4*m4*(2*cz4*c4^2 + 2*cz4*s4^2) - 2*c4*cz4*m4*(c4*cx4 - cy4*s4)) + 2*cy3*cz3*m3 + d3*m4*(2*cz4*c4^2 + 2*cz4*s4^2)) + c2*(2*c4*(Ixy4*c4 - Ixx4*s4) - 2*Ixz3 + 2*s4*(Iyy4*c4 - Ixy4*s4) - d3*(2*c3*c4*m4*(c4*cx4 - cy4*s4) + 2*m4*s3*s4*(c4*cx4 - cy4*s4)) - 2*cx3*cz3*m3 + 2*c4*cy4*m4*(c4*cx4 - cy4*s4) + 2*cx4*m4*s4*(c4*cx4 - cy4*s4))))/2 + (td4^2*(s2*(c3*(2*Iyz4 + 2*cy4*cz4*m4) + s3*(2*Ixz4 + 2*cx4*cz4*m4)) - c2*d3*(2*c3*cx4*m4 - 2*cy4*m4*s3)))/2 + (td1^2*(s2*(2*c2*(Iyz3*c2 + Ixy3*c3*s2 + Iyy3*s2*s3) - c3*(2*(c2*c4 + c3*s2*s4)*(Ixz4*(c2*s4 - c3*c4*s2) + Iyz4*(c2*c4 + c3*s2*s4) - Izz4*s2*s3) + cy4*m4*(2*(c2*s4 - c3*c4*s2)*(cz4*(c2*s4 - c3*c4*s2) - cx4*s2*s3) + 2*(c2*c4 + c3*s2*s4)*(cz4*(c2*c4 + c3*s2*s4) - cy4*s2*s3) + 2*c2*d3*s2*s3) - 2*s2*s3*(Ixy4*(c2*s4 - c3*c4*s2) - Iyy4*(c2*c4 + c3*s2*s4) + Iyz4*s2*s3) + cz4*m4*(2*(c2*s4 - c3*c4*s2)*(cx4*(c2*c4 + c3*s2*s4) - cy4*(c2*s4 - c3*c4*s2)) + c4*(2*d3*c3^2*s2^2 + 2*d3*s2^2*s3^2) + 2*s2*s3*(cz4*(c2*c4 + c3*s2*s4) - cy4*s2*s3) - 2*c2*c3*d3*s2*s4)) - s3*(2*(c2*s4 - c3*c4*s2)*(Ixz4*(c2*s4 - c3*c4*s2) + Iyz4*(c2*c4 + c3*s2*s4) - Izz4*s2*s3) + cx4*m4*(2*(c2*s4 - c3*c4*s2)*(cz4*(c2*s4 - c3*c4*s2) - cx4*s2*s3) + 2*(c2*c4 + c3*s2*s4)*(cz4*(c2*c4 + c3*s2*s4) - cy4*s2*s3) + 2*c2*d3*s2*s3) - 2*s2*s3*(Ixy4*(c2*c4 + c3*s2*s4) - Ixx4*(c2*s4 - c3*c4*s2) + Ixz4*s2*s3) + cz4*m4*(s4*(2*d3*c3^2*s2^2 + 2*d3*s2^2*s3^2) - 2*(c2*c4 + c3*s2*s4)*(cx4*(c2*c4 + c3*s2*s4) - cy4*(c2*s4 - c3*c4*s2)) + 2*s2*s3*(cz4*(c2*s4 - c3*c4*s2) - cx4*s2*s3) + 2*c2*c3*c4*d3*s2)) + cz3*m3*(2*c2*(c2*cy3 + cz3*s2*s3) + 2*c3*s2*(c3*cy3*s2 + cx3*s2*s3)) + cy3*m3*(2*c3*s2*(c2*cx3 - c3*cz3*s2) - 2*s2*s3*(c2*cy3 + cz3*s2*s3)) + d3*m4*(2*(c2*s4 - c3*c4*s2)*(cz4*(c2*s4 - c3*c4*s2) - cx4*s2*s3) + 2*(c2*c4 + c3*s2*s4)*(cz4*(c2*c4 + c3*s2*s4) - cy4*s2*s3) + 2*c2*d3*s2*s3) - 2*s2*s3*(Izz3*c2 - Ixz3*c3*s2 + Iyz3*s2*s3)) + 2*c2*(Ixy2*c2 - Ixx2*s2) + 2*s2*(Iyy2*c2 - Ixy2*s2) - c2*(2*(c2*s4 - c3*c4*s2)*(Ixy4*(c2*s4 - c3*c4*s2) - Iyy4*(c2*c4 + c3*s2*s4) + Iyz4*s2*s3) - 2*(c2*c4 + c3*s2*s4)*(Ixy4*(c2*c4 + c3*s2*s4) - Ixx4*(c2*s4 - c3*c4*s2) + Ixz4*s2*s3) - d3*(c3*m4*(s4*(2*d3*c3^2*s2^2 + 2*d3*s2^2*s3^2) - 2*(c2*c4 + c3*s2*s4)*(cx4*(c2*c4 + c3*s2*s4) - cy4*(c2*s4 - c3*c4*s2)) + 2*s2*s3*(cz4*(c2*s4 - c3*c4*s2) - cx4*s2*s3) + 2*c2*c3*c4*d3*s2) - m4*s3*(2*(c2*s4 - c3*c4*s2)*(cx4*(c2*c4 + c3*s2*s4) - cy4*(c2*s4 - c3*c4*s2)) + c4*(2*d3*c3^2*s2^2 + 2*d3*s2^2*s3^2) + 2*s2*s3*(cz4*(c2*c4 + c3*s2*s4) - cy4*s2*s3) - 2*c2*c3*d3*s2*s4)) - 2*c2*(Ixx3*c3*s2 - Ixz3*c2 + Ixy3*s2*s3) + cx3*m3*(2*c3*s2*(c2*cx3 - c3*cz3*s2) - 2*s2*s3*(c2*cy3 + cz3*s2*s3)) + cz3*m3*(2*c2*(c2*cx3 - c3*cz3*s2) + 2*s2*s3*(c3*cy3*s2 + cx3*s2*s3)) + 2*c3*s2*(Izz3*c2 - Ixz3*c3*s2 + Iyz3*s2*s3) - cx4*m4*(2*(c2*s4 - c3*c4*s2)*(cx4*(c2*c4 + c3*s2*s4) - cy4*(c2*s4 - c3*c4*s2)) + c4*(2*d3*c3^2*s2^2 + 2*d3*s2^2*s3^2) + 2*s2*s3*(cz4*(c2*c4 + c3*s2*s4) - cy4*s2*s3) - 2*c2*c3*d3*s2*s4) + cy4*m4*(s4*(2*d3*c3^2*s2^2 + 2*d3*s2^2*s3^2) - 2*(c2*c4 + c3*s2*s4)*(cx4*(c2*c4 + c3*s2*s4) - cy4*(c2*s4 - c3*c4*s2)) + 2*s2*s3*(cz4*(c2*s4 - c3*c4*s2) - cx4*s2*s3) + 2*c2*c3*c4*d3*s2)) + 2*c2*cy2*m2*(c2*cx2 - cy2*s2) + 2*cx2*m2*s2*(c2*cx2 - cy2*s2)))/2 - td2*td4*(s2*(s3*(2*Ixz4*c3 - Ixx4*c4*s3 + Iyy4*c4*s3 + Izz4*c4*s3 - 2*Ixy4*s3*s4 + cx4*m4*(2*c4*cx4*s3 - 2*cy4*s3*s4) + 2*c3*cx4*cz4*m4) + c3*(2*Iyz4*c3 + 2*Ixy4*c4*s3 - Ixx4*s3*s4 + Iyy4*s3*s4 - Izz4*s3*s4 + cy4*m4*(2*c4*cx4*s3 - 2*cy4*s3*s4) + 2*c3*cy4*cz4*m4) - d3*m4*(2*c4*cx4*s3 - 2*cy4*s3*s4)) - c2*d3*(2*c3^2*cx4*m4 - 2*c3*cy4*m4*s3)) - td1*td3*(c2*(2*Ixz3*c2 - (c2*c4 + c3*s2*s4)*(Ixy4*c4 - Ixx4*s4) - (c2*s4 - c3*c4*s2)*(Iyy4*c4 - Ixy4*s4) + d3*(c3*m4*(c4*(cx4*(c2*c4 + c3*s2*s4) - cy4*(c2*s4 - c3*c4*s2)) + (c2*c4 + c3*s2*s4)*(c4*cx4 - cy4*s4) - c3*cy4*s2 - 2*cz4*s2*s3*s4) + m4*s3*(s4*(cx4*(c2*c4 + c3*s2*s4) - cy4*(c2*s4 - c3*c4*s2)) + (c2*s4 - c3*c4*s2)*(c4*cx4 - cy4*s4) - c3*cx4*s2 + 2*c4*cz4*s2*s3)) - c4*(Ixy4*(c2*c4 + c3*s2*s4) - Ixx4*(c2*s4 - c3*c4*s2) + Ixz4*s2*s3) + s4*(Ixy4*(c2*s4 - c3*c4*s2) - Iyy4*(c2*c4 + c3*s2*s4) + Iyz4*s2*s3) - Ixx3*c3*s2 + Iyy3*c3*s2 + Izz3*c3*s2 + Izz4*c3*s2 - cx4*m4*(s4*(cx4*(c2*c4 + c3*s2*s4) - cy4*(c2*s4 - c3*c4*s2)) + (c2*s4 - c3*c4*s2)*(c4*cx4 - cy4*s4) - c3*cx4*s2 + 2*c4*cz4*s2*s3) - cy4*m4*(c4*(cx4*(c2*c4 + c3*s2*s4) - cy4*(c2*s4 - c3*c4*s2)) + (c2*c4 + c3*s2*s4)*(c4*cx4 - cy4*s4) - c3*cy4*s2 - 2*cz4*s2*s3*s4) - 2*Ixy3*s2*s3 + cx3*m3*(2*c3*cx3*s2 - 2*cy3*s2*s3) + Iyz4*s2*s3*s4 - Ixz4*c4*s2*s3 + 2*c2*cx3*cz3*m3) - s2*(2*Iyz3*c2 - c3*((c2*c4 + c3*s2*s4)*(Iyz4*c4 + Ixz4*s4) + c4*(Ixz4*(c2*s4 - c3*c4*s2) + Iyz4*(c2*c4 + c3*s2*s4) - Izz4*s2*s3) - Ixz4*c3*s2 + cz4*m4*(s4*(cx4*(c2*c4 + c3*s2*s4) - cy4*(c2*s4 - c3*c4*s2)) + (c2*s4 - c3*c4*s2)*(c4*cx4 - cy4*s4) - c3*cx4*s2 + 2*c4*cz4*s2*s3) + s2*s3*(Iyy4*c4 - Ixy4*s4) + cy4*m4*(c4*(cz4*(c2*c4 + c3*s2*s4) - cy4*s2*s3) + s4*(cz4*(c2*s4 - c3*c4*s2) - cx4*s2*s3) + c4*cz4*(c2*c4 + c3*s2*s4) + cz4*s4*(c2*s4 - c3*c4*s2) + c4*cy4*s2*s3 + cx4*s2*s3*s4) + Ixy4*s2*s3*s4 + Ixx4*c4*s2*s3) - s3*((c2*s4 - c3*c4*s2)*(Iyz4*c4 + Ixz4*s4) + s4*(Ixz4*(c2*s4 - c3*c4*s2) + Iyz4*(c2*c4 + c3*s2*s4) - Izz4*s2*s3) + Iyz4*c3*s2 - cz4*m4*(c4*(cx4*(c2*c4 + c3*s2*s4) - cy4*(c2*s4 - c3*c4*s2)) + (c2*c4 + c3*s2*s4)*(c4*cx4 - cy4*s4) - c3*cy4*s2 - 2*cz4*s2*s3*s4) - s2*s3*(Ixy4*c4 - Ixx4*s4) + cx4*m4*(c4*(cz4*(c2*c4 + c3*s2*s4) - cy4*s2*s3) + s4*(cz4*(c2*s4 - c3*c4*s2) - cx4*s2*s3) + c4*cz4*(c2*c4 + c3*s2*s4) + cz4*s4*(c2*s4 - c3*c4*s2) + c4*cy4*s2*s3 + cx4*s2*s3*s4) + Iyy4*s2*s3*s4 + Ixy4*c4*s2*s3) + 2*Ixy3*c3*s2 - Ixx3*s2*s3 + Iyy3*s2*s3 - Izz3*s2*s3 + cy3*m3*(2*c3*cx3*s2 - 2*cy3*s2*s3) + d3*m4*(c4*(cz4*(c2*c4 + c3*s2*s4) - cy4*s2*s3) + s4*(cz4*(c2*s4 - c3*c4*s2) - cx4*s2*s3) + c4*cz4*(c2*c4 + c3*s2*s4) + cz4*s4*(c2*s4 - c3*c4*s2) + c4*cy4*s2*s3 + cx4*s2*s3*s4) + 2*c2*cy3*cz3*m3)) - td1*td4*(s2*(s3*(2*Ixy4*(c2*c4 + c3*s2*s4) - Ixx4*(c2*s4 - c3*c4*s2) + Iyy4*(c2*s4 - c3*c4*s2) + Izz4*(c2*s4 - c3*c4*s2) + cx4*m4*(2*cx4*(c2*s4 - c3*c4*s2) + 2*cy4*(c2*c4 + c3*s2*s4)) + 2*Ixz4*s2*s3 + 2*cx4*cz4*m4*s2*s3) + c3*(Ixx4*(c2*c4 + c3*s2*s4) + 2*Ixy4*(c2*s4 - c3*c4*s2) - Iyy4*(c2*c4 + c3*s2*s4) + Izz4*(c2*c4 + c3*s2*s4) + cy4*m4*(2*cx4*(c2*s4 - c3*c4*s2) + 2*cy4*(c2*c4 + c3*s2*s4)) + 2*Iyz4*s2*s3 + 2*cy4*cz4*m4*s2*s3) - d3*m4*(2*cx4*(c2*s4 - c3*c4*s2) + 2*cy4*(c2*c4 + c3*s2*s4))) + c2*d3*(2*cy4*m4*s2*s3^2 - 2*c3*cx4*m4*s2*s3)) - td2*td3*(s2*(Ixx3*c3 - Iyy3*c3 + Izz3*c3 + 2*Ixy3*s3 + c3*(Ixz4*s3 - c4*(Izz4*c3 - Ixz4*c4*s3 + Iyz4*s3*s4) + c3*(Iyy4*c4 - Ixy4*s4) + Ixx4*c3*c4 + Ixy4*c3*s4 - cy4*m4*(s4*(c3*cx4 - c4*cz4*s3) + c4*(c3*cy4 + cz4*s3*s4) - c3*c4*cy4 - c3*cx4*s4) + cz4*m4*(cx4*s3 - s4*(c4*cy4*s3 + cx4*s3*s4) + 2*c3*c4*cz4 + c4*s3*(c4*cx4 - cy4*s4)) - s3*s4*(Iyz4*c4 + Ixz4*s4)) - s3*(Iyz4*s3 + c3*(Ixy4*c4 - Ixx4*s4) + s4*(Izz4*c3 - Ixz4*c4*s3 + Iyz4*s3*s4) - Ixy4*c3*c4 - Iyy4*c3*s4 + cx4*m4*(s4*(c3*cx4 - c4*cz4*s3) + c4*(c3*cy4 + cz4*s3*s4) - c3*c4*cy4 - c3*cx4*s4) - c4*s3*(Iyz4*c4 + Ixz4*s4) - cz4*m4*(c4*(c4*cy4*s3 + cx4*s3*s4) - cy4*s3 + s3*s4*(c4*cx4 - cy4*s4) + 2*c3*cz4*s4)) + d3*m4*(s4*(c3*cx4 - c4*cz4*s3) + c4*(c3*cy4 + cz4*s3*s4) - c3*c4*cy4 - c3*cx4*s4) + cy3*m3*(2*c3*cy3 + 2*cx3*s3)) - c2*(2*Ixy3*c3 - Ixx3*s3 + Iyy3*s3 + Izz3*s3 + Izz4*s3 - c4*(Ixx4*c4*s3 - Ixz4*c3 + Ixy4*s3*s4) - s4*(Iyz4*c3 + Ixy4*c4*s3 + Iyy4*s3*s4) - d3*(m4*s3*(cx4*s3 - s4*(c4*cy4*s3 + cx4*s3*s4) + 2*c3*c4*cz4 + c4*s3*(c4*cx4 - cy4*s4)) - c3*m4*(c4*(c4*cy4*s3 + cx4*s3*s4) - cy4*s3 + s3*s4*(c4*cx4 - cy4*s4) + 2*c3*cz4*s4)) + Ixz4*c3*c4 - Iyz4*c3*s4 + cx4*m4*(cx4*s3 - s4*(c4*cy4*s3 + cx4*s3*s4) + 2*c3*c4*cz4 + c4*s3*(c4*cx4 - cy4*s4)) + c4*s3*(Iyy4*c4 - Ixy4*s4) - cy4*m4*(c4*(c4*cy4*s3 + cx4*s3*s4) - cy4*s3 + s3*s4*(c4*cx4 - cy4*s4) + 2*c3*cz4*s4) - s3*s4*(Ixy4*c4 - Ixx4*s4) + cx3*m3*(2*c3*cy3 + 2*cx3*s3))) - td1*td2*(c2*((c2*c4 + c3*s2*s4)*(Ixx4*c4*s3 - Ixz4*c3 + Ixy4*s3*s4) + (c2*s4 - c3*c4*s2)*(Iyz4*c3 + Ixy4*c4*s3 + Iyy4*s3*s4) - d3*(m4*s3*((c2*s4 - c3*c4*s2)*(c4*cy4*s3 + cx4*s3*s4) - c3*(cz4*(c2*c4 + c3*s2*s4) - cy4*s2*s3) + cz4*(s2*s4 + c2*c3*c4) + s2*s3*(c3*cy4 + cz4*s3*s4) - c4*s3*(cx4*(c2*c4 + c3*s2*s4) - cy4*(c2*s4 - c3*c4*s2)) + c2*cx4*s3 - 2*c2*d3*s3*s4) + c3*m4*((c2*c4 + c3*s2*s4)*(c4*cy4*s3 + cx4*s3*s4) + c3*(cz4*(c2*s4 - c3*c4*s2) - cx4*s2*s3) + cz4*(c4*s2 - c2*c3*s4) - s2*s3*(c3*cx4 - c4*cz4*s3) + s3*s4*(cx4*(c2*c4 + c3*s2*s4) - cy4*(c2*s4 - c3*c4*s2)) + c2*cy4*s3 - 2*c2*c4*d3*s3)) - Iyz3*s2 - c2*(Ixy3*c3 - Ixx3*s3) - s3*(Izz3*c2 - Ixz3*c3*s2 + Iyz3*s2*s3) + Ixz4*(s2*s4 + c2*c3*c4) + Iyz4*(c4*s2 - c2*c3*s4) + Ixy3*c2*c3 + Iyy3*c2*s3 + Izz4*c2*s3 - cx3*m3*(s3*(c2*cx3 - c3*cz3*s2) + c3*(c2*cy3 + cz3*s2*s3) - c2*c3*cy3 - c2*cx3*s3) + c3*s2*(Iyz3*c3 + Ixz3*s3) + cz3*m3*(c3*(c3*cy3*s2 + cx3*s2*s3) - cy3*s2 + s2*s3*(c3*cx3 - cy3*s3) + 2*c2*cz3*s3) + c4*s3*(Ixy4*(c2*s4 - c3*c4*s2) - Iyy4*(c2*c4 + c3*s2*s4) + Iyz4*s2*s3) + s3*s4*(Ixy4*(c2*c4 + c3*s2*s4) - Ixx4*(c2*s4 - c3*c4*s2) + Ixz4*s2*s3) + cy4*m4*((c2*c4 + c3*s2*s4)*(c4*cy4*s3 + cx4*s3*s4) + c3*(cz4*(c2*s4 - c3*c4*s2) - cx4*s2*s3) + cz4*(c4*s2 - c2*c3*s4) - s2*s3*(c3*cx4 - c4*cz4*s3) + s3*s4*(cx4*(c2*c4 + c3*s2*s4) - cy4*(c2*s4 - c3*c4*s2)) + c2*cy4*s3 - 2*c2*c4*d3*s3) + cx4*m4*((c2*s4 - c3*c4*s2)*(c4*cy4*s3 + cx4*s3*s4) - c3*(cz4*(c2*c4 + c3*s2*s4) - cy4*s2*s3) + cz4*(s2*s4 + c2*c3*c4) + s2*s3*(c3*cy4 + cz4*s3*s4) - c4*s3*(cx4*(c2*c4 + c3*s2*s4) - cy4*(c2*s4 - c3*c4*s2)) + c2*cx4*s3 - 2*c2*d3*s3*s4)) - s2*(c3*((c2*c4 + c3*s2*s4)*(Izz4*c3 - Ixz4*c4*s3 + Iyz4*s3*s4) + c3*(Ixy4*(c2*s4 - c3*c4*s2) - Iyy4*(c2*c4 + c3*s2*s4) + Iyz4*s2*s3) + Ixx4*(s2*s4 + c2*c3*c4) - Ixy4*(c4*s2 - c2*c3*s4) + Ixz4*c2*s3 + s2*s3*(Iyz4*c3 + Ixy4*c4*s3 + Iyy4*s3*s4) + cy4*m4*((c3*cx4 - c4*cz4*s3)*(c2*s4 - c3*c4*s2) + (c2*c4 + c3*s2*s4)*(c3*cy4 + cz4*s3*s4) - cx4*(c4*s2 - c2*c3*s4) + cy4*(s2*s4 + c2*c3*c4) - c4*s3*(cz4*(c2*s4 - c3*c4*s2) - cx4*s2*s3) + s3*s4*(cz4*(c2*c4 + c3*s2*s4) - cy4*s2*s3) - 2*c2*c3*d3) + s3*s4*(Ixz4*(c2*s4 - c3*c4*s2) + Iyz4*(c2*c4 + c3*s2*s4) - Izz4*s2*s3) + cz4*m4*((c2*s4 - c3*c4*s2)*(c4*cy4*s3 + cx4*s3*s4) - c3*(cz4*(c2*c4 + c3*s2*s4) - cy4*s2*s3) + cz4*(s2*s4 + c2*c3*c4) + s2*s3*(c3*cy4 + cz4*s3*s4) - c4*s3*(cx4*(c2*c4 + c3*s2*s4) - cy4*(c2*s4 - c3*c4*s2)) + c2*cx4*s3 - 2*c2*d3*s3*s4)) - s3*(Iyy4*(c4*s2 - c2*c3*s4) - c3*(Ixy4*(c2*c4 + c3*s2*s4) - Ixx4*(c2*s4 - c3*c4*s2) + Ixz4*s2*s3) - Ixy4*(s2*s4 + c2*c3*c4) - (c2*s4 - c3*c4*s2)*(Izz4*c3 - Ixz4*c4*s3 + Iyz4*s3*s4) + Iyz4*c2*s3 + s2*s3*(Ixx4*c4*s3 - Ixz4*c3 + Ixy4*s3*s4) - cx4*m4*((c3*cx4 - c4*cz4*s3)*(c2*s4 - c3*c4*s2) + (c2*c4 + c3*s2*s4)*(c3*cy4 + cz4*s3*s4) - cx4*(c4*s2 - c2*c3*s4) + cy4*(s2*s4 + c2*c3*c4) - c4*s3*(cz4*(c2*s4 - c3*c4*s2) - cx4*s2*s3) + s3*s4*(cz4*(c2*c4 + c3*s2*s4) - cy4*s2*s3) - 2*c2*c3*d3) + c4*s3*(Ixz4*(c2*s4 - c3*c4*s2) + Iyz4*(c2*c4 + c3*s2*s4) - Izz4*s2*s3) + cz4*m4*((c2*c4 + c3*s2*s4)*(c4*cy4*s3 + cx4*s3*s4) + c3*(cz4*(c2*s4 - c3*c4*s2) - cx4*s2*s3) + cz4*(c4*s2 - c2*c3*s4) - s2*s3*(c3*cx4 - c4*cz4*s3) + s3*s4*(cx4*(c2*c4 + c3*s2*s4) - cy4*(c2*s4 - c3*c4*s2)) + c2*cy4*s3 - 2*c2*c4*d3*s3)) + Ixz3*s2 - c3*(Izz3*c2 - Ixz3*c3*s2 + Iyz3*s2*s3) + c2*(Iyy3*c3 - Ixy3*s3) + Ixx3*c2*c3 + Ixy3*c2*s3 - cy3*m3*(s3*(c2*cx3 - c3*cz3*s2) + c3*(c2*cy3 + cz3*s2*s3) - c2*c3*cy3 - c2*cx3*s3) + cz3*m3*(cx3*s2 - s3*(c3*cy3*s2 + cx3*s2*s3) + 2*c2*c3*cz3 + c3*s2*(c3*cx3 - cy3*s3)) - d3*m4*((c3*cx4 - c4*cz4*s3)*(c2*s4 - c3*c4*s2) + (c2*c4 + c3*s2*s4)*(c3*cy4 + cz4*s3*s4) - cx4*(c4*s2 - c2*c3*s4) + cy4*(s2*s4 + c2*c3*c4) - c4*s3*(cz4*(c2*s4 - c3*c4*s2) - cx4*s2*s3) + s3*s4*(cz4*(c2*c4 + c3*s2*s4) - cy4*s2*s3) - 2*c2*c3*d3) - s2*s3*(Iyz3*c3 + Ixz3*s3))) - s2*td3*td4*(c3*(Ixx4*c4 - Iyy4*c4 + Izz4*c4 + 2*Ixy4*s4 + cy4*m4*(2*c4*cy4 + 2*cx4*s4)) + s3*(2*Ixy4*c4 - Ixx4*s4 + Iyy4*s4 + Izz4*s4 + cx4*m4*(2*c4*cy4 + 2*cx4*s4)) - d3*m4*(2*c4*cy4 + 2*cx4*s4));
corio3 = (td2^2*(c3*(cx4*m4*(2*c4*s3*(c3*cx4 - c4*cz4*s3) - 2*s3*s4*(c3*cy4 + cz4*s3*s4)) - 2*c3*(Ixx4*c4*s3 - Ixz4*c3 + Ixy4*s3*s4) + cz4*m4*(2*c3*(c3*cx4 - c4*cz4*s3) - s4*(2*d3*c3^2 + 2*d3*s3^2) + 2*s3*s4*(c4*cy4*s3 + cx4*s3*s4)) + 2*c4*s3*(Izz4*c3 - Ixz4*c4*s3 + Iyz4*s3*s4)) - s3*(2*c3*(Iyz4*c3 + Ixy4*c4*s3 + Iyy4*s3*s4) + cy4*m4*(2*c4*s3*(c3*cx4 - c4*cz4*s3) - 2*s3*s4*(c3*cy4 + cz4*s3*s4)) + cz4*m4*(2*c3*(c3*cy4 + cz4*s3*s4) - c4*(2*d3*c3^2 + 2*d3*s3^2) + 2*c4*s3*(c4*cy4*s3 + cx4*s3*s4)) - 2*s3*s4*(Izz4*c3 - Ixz4*c4*s3 + Iyz4*s3*s4)) + 2*c3*(Ixy3*c3 - Ixx3*s3) + 2*s3*(Iyy3*c3 - Ixy3*s3) + 2*c3*cy3*m3*(c3*cx3 - cy3*s3) + 2*cx3*m3*s3*(c3*cx3 - cy3*s3)))/2 - (td1^2*(c3*(2*(c2*s4 - c3*c4*s2)*(Ixz4*(c2*s4 - c3*c4*s2) + Iyz4*(c2*c4 + c3*s2*s4) - Izz4*s2*s3) + cx4*m4*(2*(c2*s4 - c3*c4*s2)*(cz4*(c2*s4 - c3*c4*s2) - cx4*s2*s3) + 2*(c2*c4 + c3*s2*s4)*(cz4*(c2*c4 + c3*s2*s4) - cy4*s2*s3) + 2*c2*d3*s2*s3) - 2*s2*s3*(Ixy4*(c2*c4 + c3*s2*s4) - Ixx4*(c2*s4 - c3*c4*s2) + Ixz4*s2*s3) + cz4*m4*(s4*(2*d3*c3^2*s2^2 + 2*d3*s2^2*s3^2) - 2*(c2*c4 + c3*s2*s4)*(cx4*(c2*c4 + c3*s2*s4) - cy4*(c2*s4 - c3*c4*s2)) + 2*s2*s3*(cz4*(c2*s4 - c3*c4*s2) - cx4*s2*s3) + 2*c2*c3*c4*d3*s2)) - s3*(2*(c2*c4 + c3*s2*s4)*(Ixz4*(c2*s4 - c3*c4*s2) + Iyz4*(c2*c4 + c3*s2*s4) - Izz4*s2*s3) + cy4*m4*(2*(c2*s4 - c3*c4*s2)*(cz4*(c2*s4 - c3*c4*s2) - cx4*s2*s3) + 2*(c2*c4 + c3*s2*s4)*(cz4*(c2*c4 + c3*s2*s4) - cy4*s2*s3) + 2*c2*d3*s2*s3) - 2*s2*s3*(Ixy4*(c2*s4 - c3*c4*s2) - Iyy4*(c2*c4 + c3*s2*s4) + Iyz4*s2*s3) + cz4*m4*(2*(c2*s4 - c3*c4*s2)*(cx4*(c2*c4 + c3*s2*s4) - cy4*(c2*s4 - c3*c4*s2)) + c4*(2*d3*c3^2*s2^2 + 2*d3*s2^2*s3^2) + 2*s2*s3*(cz4*(c2*c4 + c3*s2*s4) - cy4*s2*s3) - 2*c2*c3*d3*s2*s4)) + cx3*m3*(2*c2*(c2*cy3 + cz3*s2*s3) + 2*c3*s2*(c3*cy3*s2 + cx3*s2*s3)) - cy3*m3*(2*c2*(c2*cx3 - c3*cz3*s2) + 2*s2*s3*(c3*cy3*s2 + cx3*s2*s3)) + 2*c3*s2*(Iyz3*c2 + Ixy3*c3*s2 + Iyy3*s2*s3) - 2*s2*s3*(Ixx3*c3*s2 - Ixz3*c2 + Ixy3*s2*s3)))/2 + (td4^2*(c3*(2*Ixz4 + 2*cx4*cz4*m4) - s3*(2*Iyz4 + 2*cy4*cz4*m4)))/2 - (td3^2*(c3*(2*s4*(Iyz4*c4 + Ixz4*s4) + cx4*m4*(2*cz4*c4^2 + 2*cz4*s4^2) - 2*c4*cz4*m4*(c4*cx4 - cy4*s4)) - s3*(2*c4*(Iyz4*c4 + Ixz4*s4) + cy4*m4*(2*cz4*c4^2 + 2*cz4*s4^2) + 2*cz4*m4*s4*(c4*cx4 - cy4*s4))))/2 - td1*td2*(Izz3*s2 + s3*((c2*c4 + c3*s2*s4)*(Izz4*c3 - Ixz4*c4*s3 + Iyz4*s3*s4) + c3*(Ixy4*(c2*s4 - c3*c4*s2) - Iyy4*(c2*c4 + c3*s2*s4) + Iyz4*s2*s3) + Ixx4*(s2*s4 + c2*c3*c4) - Ixy4*(c4*s2 - c2*c3*s4) + Ixz4*c2*s3 + s2*s3*(Iyz4*c3 + Ixy4*c4*s3 + Iyy4*s3*s4) + cy4*m4*((c3*cx4 - c4*cz4*s3)*(c2*s4 - c3*c4*s2) + (c2*c4 + c3*s2*s4)*(c3*cy4 + cz4*s3*s4) - cx4*(c4*s2 - c2*c3*s4) + cy4*(s2*s4 + c2*c3*c4) - c4*s3*(cz4*(c2*s4 - c3*c4*s2) - cx4*s2*s3) + s3*s4*(cz4*(c2*c4 + c3*s2*s4) - cy4*s2*s3) - 2*c2*c3*d3) + s3*s4*(Ixz4*(c2*s4 - c3*c4*s2) + Iyz4*(c2*c4 + c3*s2*s4) - Izz4*s2*s3) + cz4*m4*((c2*s4 - c3*c4*s2)*(c4*cy4*s3 + cx4*s3*s4) - c3*(cz4*(c2*c4 + c3*s2*s4) - cy4*s2*s3) + cz4*(s2*s4 + c2*c3*c4) + s2*s3*(c3*cy4 + cz4*s3*s4) - c4*s3*(cx4*(c2*c4 + c3*s2*s4) - cy4*(c2*s4 - c3*c4*s2)) + c2*cx4*s3 - 2*c2*d3*s3*s4)) - c3*(Ixx3*c3*s2 - Ixz3*c2 + Ixy3*s2*s3) - s3*(Iyz3*c2 + Ixy3*c3*s2 + Iyy3*s2*s3) + c3*(Iyy4*(c4*s2 - c2*c3*s4) - c3*(Ixy4*(c2*c4 + c3*s2*s4) - Ixx4*(c2*s4 - c3*c4*s2) + Ixz4*s2*s3) - Ixy4*(s2*s4 + c2*c3*c4) - (c2*s4 - c3*c4*s2)*(Izz4*c3 - Ixz4*c4*s3 + Iyz4*s3*s4) + Iyz4*c2*s3 + s2*s3*(Ixx4*c4*s3 - Ixz4*c3 + Ixy4*s3*s4) - cx4*m4*((c3*cx4 - c4*cz4*s3)*(c2*s4 - c3*c4*s2) + (c2*c4 + c3*s2*s4)*(c3*cy4 + cz4*s3*s4) - cx4*(c4*s2 - c2*c3*s4) + cy4*(s2*s4 + c2*c3*c4) - c4*s3*(cz4*(c2*s4 - c3*c4*s2) - cx4*s2*s3) + s3*s4*(cz4*(c2*c4 + c3*s2*s4) - cy4*s2*s3) - 2*c2*c3*d3) + c4*s3*(Ixz4*(c2*s4 - c3*c4*s2) + Iyz4*(c2*c4 + c3*s2*s4) - Izz4*s2*s3) + cz4*m4*((c2*c4 + c3*s2*s4)*(c4*cy4*s3 + cx4*s3*s4) + c3*(cz4*(c2*s4 - c3*c4*s2) - cx4*s2*s3) + cz4*(c4*s2 - c2*c3*s4) - s2*s3*(c3*cx4 - c4*cz4*s3) + s3*s4*(cx4*(c2*c4 + c3*s2*s4) - cy4*(c2*s4 - c3*c4*s2)) + c2*cy4*s3 - 2*c2*c4*d3*s3)) + Ixz3*c2*c3 - Iyz3*c2*s3 + cx3*m3*(cx3*s2 - s3*(c3*cy3*s2 + cx3*s2*s3) + 2*c2*c3*cz3 + c3*s2*(c3*cx3 - cy3*s3)) + c3*s2*(Iyy3*c3 - Ixy3*s3) - cy3*m3*(c3*(c3*cy3*s2 + cx3*s2*s3) - cy3*s2 + s2*s3*(c3*cx3 - cy3*s3) + 2*c2*cz3*s3) - s2*s3*(Ixy3*c3 - Ixx3*s3)) + td2*td3*(s3*(Ixz4*s3 - c4*(Izz4*c3 - Ixz4*c4*s3 + Iyz4*s3*s4) + c3*(Iyy4*c4 - Ixy4*s4) + Ixx4*c3*c4 + Ixy4*c3*s4 - cy4*m4*(s4*(c3*cx4 - c4*cz4*s3) + c4*(c3*cy4 + cz4*s3*s4) - c3*c4*cy4 - c3*cx4*s4) + cz4*m4*(cx4*s3 - s4*(c4*cy4*s3 + cx4*s3*s4) + 2*c3*c4*cz4 + c4*s3*(c4*cx4 - cy4*s4)) - s3*s4*(Iyz4*c4 + Ixz4*s4)) + c3*(Iyz4*s3 + c3*(Ixy4*c4 - Ixx4*s4) + s4*(Izz4*c3 - Ixz4*c4*s3 + Iyz4*s3*s4) - Ixy4*c3*c4 - Iyy4*c3*s4 + cx4*m4*(s4*(c3*cx4 - c4*cz4*s3) + c4*(c3*cy4 + cz4*s3*s4) - c3*c4*cy4 - c3*cx4*s4) - c4*s3*(Iyz4*c4 + Ixz4*s4) - cz4*m4*(c4*(c4*cy4*s3 + cx4*s3*s4) - cy4*s3 + s3*s4*(c4*cx4 - cy4*s4) + 2*c3*cz4*s4))) + td1*td3*(s3*((c2*c4 + c3*s2*s4)*(Iyz4*c4 + Ixz4*s4) + c4*(Ixz4*(c2*s4 - c3*c4*s2) + Iyz4*(c2*c4 + c3*s2*s4) - Izz4*s2*s3) - Ixz4*c3*s2 + cz4*m4*(s4*(cx4*(c2*c4 + c3*s2*s4) - cy4*(c2*s4 - c3*c4*s2)) + (c2*s4 - c3*c4*s2)*(c4*cx4 - cy4*s4) - c3*cx4*s2 + 2*c4*cz4*s2*s3) + s2*s3*(Iyy4*c4 - Ixy4*s4) + cy4*m4*(c4*(cz4*(c2*c4 + c3*s2*s4) - cy4*s2*s3) + s4*(cz4*(c2*s4 - c3*c4*s2) - cx4*s2*s3) + c4*cz4*(c2*c4 + c3*s2*s4) + cz4*s4*(c2*s4 - c3*c4*s2) + c4*cy4*s2*s3 + cx4*s2*s3*s4) + Ixy4*s2*s3*s4 + Ixx4*c4*s2*s3) - c3*((c2*s4 - c3*c4*s2)*(Iyz4*c4 + Ixz4*s4) + s4*(Ixz4*(c2*s4 - c3*c4*s2) + Iyz4*(c2*c4 + c3*s2*s4) - Izz4*s2*s3) + Iyz4*c3*s2 - cz4*m4*(c4*(cx4*(c2*c4 + c3*s2*s4) - cy4*(c2*s4 - c3*c4*s2)) + (c2*c4 + c3*s2*s4)*(c4*cx4 - cy4*s4) - c3*cy4*s2 - 2*cz4*s2*s3*s4) - s2*s3*(Ixy4*c4 - Ixx4*s4) + cx4*m4*(c4*(cz4*(c2*c4 + c3*s2*s4) - cy4*s2*s3) + s4*(cz4*(c2*s4 - c3*c4*s2) - cx4*s2*s3) + c4*cz4*(c2*c4 + c3*s2*s4) + cz4*s4*(c2*s4 - c3*c4*s2) + c4*cy4*s2*s3 + cx4*s2*s3*s4) + Iyy4*s2*s3*s4 + Ixy4*c4*s2*s3)) + td3*td4*(s3*(Ixx4*c4 - Iyy4*c4 + Izz4*c4 + 2*Ixy4*s4 + cy4*m4*(2*c4*cy4 + 2*cx4*s4)) - c3*(2*Ixy4*c4 - Ixx4*s4 + Iyy4*s4 + Izz4*s4 + cx4*m4*(2*c4*cy4 + 2*cx4*s4))) + td1*td4*(s3*(Ixx4*(c2*c4 + c3*s2*s4) + 2*Ixy4*(c2*s4 - c3*c4*s2) - Iyy4*(c2*c4 + c3*s2*s4) + Izz4*(c2*c4 + c3*s2*s4) + cy4*m4*(2*cx4*(c2*s4 - c3*c4*s2) + 2*cy4*(c2*c4 + c3*s2*s4)) + 2*Iyz4*s2*s3 + 2*cy4*cz4*m4*s2*s3) - c3*(2*Ixy4*(c2*c4 + c3*s2*s4) - Ixx4*(c2*s4 - c3*c4*s2) + Iyy4*(c2*s4 - c3*c4*s2) + Izz4*(c2*s4 - c3*c4*s2) + cx4*m4*(2*cx4*(c2*s4 - c3*c4*s2) + 2*cy4*(c2*c4 + c3*s2*s4)) + 2*Ixz4*s2*s3 + 2*cx4*cz4*m4*s2*s3)) - td2*td4*(c3*(2*Ixz4*c3 - Ixx4*c4*s3 + Iyy4*c4*s3 + Izz4*c4*s3 - 2*Ixy4*s3*s4 + cx4*m4*(2*c4*cx4*s3 - 2*cy4*s3*s4) + 2*c3*cx4*cz4*m4) - s3*(2*Iyz4*c3 + 2*Ixy4*c4*s3 - Ixx4*s3*s4 + Iyy4*s3*s4 - Izz4*s3*s4 + cy4*m4*(2*c4*cx4*s3 - 2*cy4*s3*s4) + 2*c3*cy4*cz4*m4));
corio4 = (td1^2*(2*(c2*c4 + c3*s2*s4)*(Ixy4*(c2*c4 + c3*s2*s4) - Ixx4*(c2*s4 - c3*c4*s2) + Ixz4*s2*s3) - 2*(c2*s4 - c3*c4*s2)*(Ixy4*(c2*s4 - c3*c4*s2) - Iyy4*(c2*c4 + c3*s2*s4) + Iyz4*s2*s3) + cx4*m4*(2*(c2*s4 - c3*c4*s2)*(cx4*(c2*c4 + c3*s2*s4) - cy4*(c2*s4 - c3*c4*s2)) + c4*(2*d3*c3^2*s2^2 + 2*d3*s2^2*s3^2) + 2*s2*s3*(cz4*(c2*c4 + c3*s2*s4) - cy4*s2*s3) - 2*c2*c3*d3*s2*s4) - cy4*m4*(s4*(2*d3*c3^2*s2^2 + 2*d3*s2^2*s3^2) - 2*(c2*c4 + c3*s2*s4)*(cx4*(c2*c4 + c3*s2*s4) - cy4*(c2*s4 - c3*c4*s2)) + 2*s2*s3*(cz4*(c2*s4 - c3*c4*s2) - cx4*s2*s3) + 2*c2*c3*c4*d3*s2)))/2 - (td2^2*(cx4*m4*(2*c3*(c3*cy4 + cz4*s3*s4) - c4*(2*d3*c3^2 + 2*d3*s3^2) + 2*c4*s3*(c4*cy4*s3 + cx4*s3*s4)) - cy4*m4*(2*c3*(c3*cx4 - c4*cz4*s3) - s4*(2*d3*c3^2 + 2*d3*s3^2) + 2*s3*s4*(c4*cy4*s3 + cx4*s3*s4)) + 2*c4*s3*(Iyz4*c3 + Ixy4*c4*s3 + Iyy4*s3*s4) - 2*s3*s4*(Ixx4*c4*s3 - Ixz4*c3 + Ixy4*s3*s4)))/2 + (td3^2*(2*c4*(Ixy4*c4 - Ixx4*s4) + 2*s4*(Iyy4*c4 - Ixy4*s4) + 2*c4*cy4*m4*(c4*cx4 - cy4*s4) + 2*cx4*m4*s4*(c4*cx4 - cy4*s4)))/2 + td1*td3*((c2*c4 + c3*s2*s4)*(Ixy4*c4 - Ixx4*s4) + (c2*s4 - c3*c4*s2)*(Iyy4*c4 - Ixy4*s4) + c4*(Ixy4*(c2*c4 + c3*s2*s4) - Ixx4*(c2*s4 - c3*c4*s2) + Ixz4*s2*s3) - s4*(Ixy4*(c2*s4 - c3*c4*s2) - Iyy4*(c2*c4 + c3*s2*s4) + Iyz4*s2*s3) - Izz4*c3*s2 + cx4*m4*(s4*(cx4*(c2*c4 + c3*s2*s4) - cy4*(c2*s4 - c3*c4*s2)) + (c2*s4 - c3*c4*s2)*(c4*cx4 - cy4*s4) - c3*cx4*s2 + 2*c4*cz4*s2*s3) + cy4*m4*(c4*(cx4*(c2*c4 + c3*s2*s4) - cy4*(c2*s4 - c3*c4*s2)) + (c2*c4 + c3*s2*s4)*(c4*cx4 - cy4*s4) - c3*cy4*s2 - 2*cz4*s2*s3*s4) - Iyz4*s2*s3*s4 + Ixz4*c4*s2*s3) - td2*td3*(c4*(Ixx4*c4*s3 - Ixz4*c3 + Ixy4*s3*s4) - Izz4*s3 + s4*(Iyz4*c3 + Ixy4*c4*s3 + Iyy4*s3*s4) - Ixz4*c3*c4 + Iyz4*c3*s4 - cx4*m4*(cx4*s3 - s4*(c4*cy4*s3 + cx4*s3*s4) + 2*c3*c4*cz4 + c4*s3*(c4*cx4 - cy4*s4)) - c4*s3*(Iyy4*c4 - Ixy4*s4) + cy4*m4*(c4*(c4*cy4*s3 + cx4*s3*s4) - cy4*s3 + s3*s4*(c4*cx4 - cy4*s4) + 2*c3*cz4*s4) + s3*s4*(Ixy4*c4 - Ixx4*s4)) - td1*td2*((c2*c4 + c3*s2*s4)*(Ixx4*c4*s3 - Ixz4*c3 + Ixy4*s3*s4) + (c2*s4 - c3*c4*s2)*(Iyz4*c3 + Ixy4*c4*s3 + Iyy4*s3*s4) + Ixz4*(s2*s4 + c2*c3*c4) + Iyz4*(c4*s2 - c2*c3*s4) + Izz4*c2*s3 + c4*s3*(Ixy4*(c2*s4 - c3*c4*s2) - Iyy4*(c2*c4 + c3*s2*s4) + Iyz4*s2*s3) + s3*s4*(Ixy4*(c2*c4 + c3*s2*s4) - Ixx4*(c2*s4 - c3*c4*s2) + Ixz4*s2*s3) + cy4*m4*((c2*c4 + c3*s2*s4)*(c4*cy4*s3 + cx4*s3*s4) + c3*(cz4*(c2*s4 - c3*c4*s2) - cx4*s2*s3) + cz4*(c4*s2 - c2*c3*s4) - s2*s3*(c3*cx4 - c4*cz4*s3) + s3*s4*(cx4*(c2*c4 + c3*s2*s4) - cy4*(c2*s4 - c3*c4*s2)) + c2*cy4*s3 - 2*c2*c4*d3*s3) + cx4*m4*((c2*s4 - c3*c4*s2)*(c4*cy4*s3 + cx4*s3*s4) - c3*(cz4*(c2*c4 + c3*s2*s4) - cy4*s2*s3) + cz4*(s2*s4 + c2*c3*c4) + s2*s3*(c3*cy4 + cz4*s3*s4) - c4*s3*(cx4*(c2*c4 + c3*s2*s4) - cy4*(c2*s4 - c3*c4*s2)) + c2*cx4*s3 - 2*c2*d3*s3*s4));

V = [corio1;
     corio2;
     corio3;
     corio4];
 
  %% matrix G
 
 g1 = g*(s2*(c3*(cz4*m4*(c2*c4 + c3*s2*s4) - cy4*m4*s2*s3) + s3*(cz4*m4*(c2*s4 - c3*c4*s2) - cx4*m4*s2*s3) + c2*cy3*m3 + cz3*m3*s2*s3 + d3*m4*s2*s3) - c2*(d3*(c3*m4*(c2*s4 - c3*c4*s2) - m4*s3*(c2*c4 + c3*s2*s4)) + cx4*m4*(c2*c4 + c3*s2*s4) - cy4*m4*(c2*s4 - c3*c4*s2) + c2*cx3*m3 - c3*cz3*m3*s2) + c2*cx2*m2 - cy2*m2*s2);
 g2 = g*(s2*(c3*(cz4*m4*(c2*c4 + c3*s2*s4) - cy4*m4*s2*s3) + s3*(cz4*m4*(c2*s4 - c3*c4*s2) - cx4*m4*s2*s3) + c2*cy3*m3 + cz3*m3*s2*s3 + d3*m4*s2*s3) - c2*(d3*(c3*m4*(c2*s4 - c3*c4*s2) - m4*s3*(c2*c4 + c3*s2*s4)) + cx4*m4*(c2*c4 + c3*s2*s4) - cy4*m4*(c2*s4 - c3*c4*s2) + c2*cx3*m3 - c3*cz3*m3*s2) + c2*cx2*m2 - cy2*m2*s2);
 g3 = -g*(s3*(cz4*m4*(c2*c4 + c3*s2*s4) - cy4*m4*s2*s3) - c3*(cz4*m4*(c2*s4 - c3*c4*s2) - cx4*m4*s2*s3) + c3*cy3*m3*s2 + cx3*m3*s2*s3);
 g4 = -g*(cx4*m4*(c2*c4 + c3*s2*s4) - cy4*m4*(c2*s4 - c3*c4*s2));
 
 G = [g1;
     g2;
     g3;
     g4];
 
 %% Controller
Kp = 10;
Kd = 10;
Ki = 1;
 
%% out put

a = q_des_ddot - Kp*(q - q_des) - Kd*(q_dot - q_des_dot) - Ki*e_int;
torque = M*a + V + G;
